simulink model "SIM_EXO_DAL"  (R2021b)
settings: Solver=VariableStepAuto  StartTime=0.0  StopTime=60  FixedStep=0.0001  RelTol=1e-4
undefined symbols (not defined in the file): b, dq, q, X, Y, Z
libraries: sm_lib x47, nesl_utility x7
(part 20 of 25)

== matlab function SIM_EXO_DAL/Energy Analysis/K ==
  data: q input; dq input; K output
function K = K(q,dq)
%#codegen
dq1 = dq(1);
dq2 = dq(2);
dq3 = dq(3);
dq4 = dq(4);
dq5 = dq(5);
dq6 = dq(6);

q1 = q(1);
q2 = q(2);
q3 = q(3);
q4 = q(4);
q5 = q(5);
q6 = q(6);
%    This function was generated by the Symbolic Math Toolbox version 9.0.
%    02-Dec-2021 21:08:55

t2 = cos(q2);
t3 = cos(q4);
t4 = cos(q5);
t5 = cos(q6);
t6 = sin(q2);
t7 = sin(q4);
t8 = sin(q5);
t9 = sin(q6);
t10 = q1+q2;
t11 = q4.*2.0;
t12 = q5.*2.0;
t13 = q6.*2.0;
t30 = 9.007199254740992e+15;
t14 = cos(t12);
t15 = cos(t13);
t16 = t3.^2;
t17 = t4.^2;
t18 = t5.^2;
t19 = sin(t11);
t20 = sin(t12);
t21 = sin(t13);
t22 = cos(t10);
t23 = sin(t10);
t29 = t8.*5.110348748545983e-1;
t31 = t4.*t5.*5.110348748545983e-1;
t32 = t4.*t9.*5.110348748545983e-1;
t33 = t4.*t7.*8.595599785252598e-1;
t34 = t3.*t9.*8.595599785252598e-1;
t35 = t5.*1.33637579258949e-4;
t37 = t3.*t5.*8.595599785252598e-1;
t38 = t9.*7.26350610236655e-5;
t39 = t5.*t7.*t8.*8.595599785252598e-1;
t40 = t7.*t8.*t9.*8.595599785252598e-1;
t41 = t9.*1.744166498897461e-6;
t42 = t5.*1.246862701090643e-6;
t43 = t9.*1.246862701090643e-6;
t44 = t8.*4.20092050615074e-6;
t45 = t5.*3.383302988283333e-6;
t51 = t4.*t9.*3.383302988283333e-6;
t52 = t8.*1.758766830582798e-8;
t53 = t4.*t5.*1.744166498897461e-6;
t54 = t5.*t8.*8.01825475553694e-7;
t55 = t4.*t5.*(-1.246862701090643e-6);
t56 = t4.*t9.*(-1.246862701090643e-6);
t57 = t4.*2.524706033578261e-9;
t58 = t8.*t9.*4.35810366141993e-7;
t59 = t5.*3.146556677756745e-13;
t60 = t8.*3.146556677756745e-13;
t61 = t8.*4.126305279697715e-13;
t62 = t9.*4.126305279697715e-13;
t63 = t4.*t9.*3.146556677756745e-13;
t65 = t4.*t5.*4.126305279697715e-13;
t66 = t5.*t8.*8.4155913e-14;
t67 = t8.*t9.*8.4155913e-14;
t68 = (q3.*t30)./4.503599627370496e+15;
t70 = (q3.*t30)./9.007199254740992e+15;
t78 = t8.*6.829346359246847e-5;
t82 = t3.*5.316841594276996e-5;
t83 = t4.*6.932317328700695e-5;
t84 = t3.*1.166014850920627e-4;
t85 = t3.*t5.*1.148695147579899e-4;
t86 = t8.*3.161026044296245e-5;
t87 = t4.*t9.*6.829346359246847e-5;
t88 = t4.*t7.*1.148695147579899e-4;
t89 = t8.*3.711904932028501e-5;
t90 = t8.*2.146816885134859e-6;
t91 = t8.*3.004073648334264e-7;
t93 = t4.*3.726186752973823e-7;
t94 = t8.*3.726186752973823e-7;
t95 = t4.*t7.*5.316841594276996e-5;
t97 = t4.*3.60334715805357e-7;
t98 = t8.*3.60334715805357e-7;
t99 = t4.*1.153569201933121e-6;
t100 = t7.*t8.*1.166014850920627e-4;
t101 = t3.*2.28624364216682e-6;
t102 = t8.*8.987911871652987e-9;
t103 = t4.*t5.*3.711904932028501e-5;
t104 = t7.*t8.*t9.*1.148695147579899e-4;
t106 = t4.*t7.*6.243419149368285e-5;
t107 = t3.*t9.*6.243419149368285e-5;
t108 = t4.*t5.*8.913299084896471e-7;
t115 = t4.*t9.*1.728985819212562e-6;
t116 = t4.*t5.*6.371903244127231e-7;
t117 = t4.*t9.*6.371903244127231e-7;
t118 = t7.*t8.*1.940301860461398e-6;
t119 = t4.*t7.*3.610943140053254e-6;
t120 = t3.*t5.*2.908151843953269e-6;
t122 = t4.*t7.*5.052847873416058e-7;
t123 = t3.*t5.*1.07175327657342e-6;
t124 = t3.*t9.*1.07175327657342e-6;
t125 = t3.*t9.*1.49921571833678e-6;
t126 = t4.*t7.*6.267441153167058e-7;
t127 = t7.*t8.*6.267441153167058e-7;
t128 = t3.*1.511765579126689e-8;
t129 = t4.*t7.*6.060825118201251e-7;
t131 = t7.*t8.*6.060825118201251e-7;
t134 = t4.*1.290212831914316e-9;
t135 = t8.*1.608000198040319e-13;
t137 = t3.*2.170136264005124e-9;
t140 = t5.*t7.*t8.*6.243419149368285e-5;
t141 = t3.*t4.*t9.*6.892170885479394e-7;
t143 = t7.*t8.*t9.*2.908151843953269e-6;
t144 = t5.*t7.*t8.*1.07175327657342e-6;
t146 = t7.*t8.*t9.*1.07175327657342e-6;
t147 = t5.*t7.*t8.*1.49921571833678e-6;
t149 = t4.*t7.*1.511765579126689e-8;
t150 = t4.*t9.*1.608000198040319e-13;
t153 = t7.*t8.*2.170136264005124e-9;
t154 = t3.*t8.*(-1.511765579126689e-8);
t157 = t3.*t4.*t5.*3.746051489620971e-7;
t158 = t4.*t5.*7.16776774470491e-12;
t159 = t4.*t9.*7.16776774470491e-12;
t160 = t8.*2.10868590222219e-13;
t161 = t3.*t5.*2.7046541903611e-13;
t162 = t4.*t7.*2.7046541903611e-13;
t164 = t3.*t5.*1.205617579517561e-11;
t165 = t3.*t9.*1.205617579517561e-11;
t167 = t4.*t7.*3.546806877605634e-13;
t168 = t3.*t9.*3.546806877605634e-13;
t169 = t4.*t5.*2.10868590222219e-13;
t172 = t7.*t8.*t9.*2.7046541903611e-13;
t173 = t5.*t7.*t8.*1.205617579517561e-11;
t174 = t7.*t8.*t9.*1.205617579517561e-11;
t177 = t5.*t7.*t8.*3.546806877605634e-13;
t180 = t3.*t8.*t9.*(-3.546806877605634e-13);
t192 = t3.*2.625549359694895e-3;
t193 = t4.*1.560969940408669e-3;
t194 = t8.*1.560969940408669e-3;
t195 = t6.*t8.*1.324388487819695e-2;
t196 = t2.*t8.*5.463144604697158e-2;
t202 = t4.*t7.*2.625549359694895e-3;
t204 = t7.*t8.*2.625549359694895e-3;
t207 = t4.*t6.*t7.*2.227619671697157e-2;
t208 = t7.*5.363539617571206e-4;
t209 = t3.*t5.*(-2.625549359694895e-3);
t210 = t4.*t5.*(-1.560969940408669e-3);
t211 = t4.*t9.*(-1.560969940408669e-3);
t217 = t2.*t4.*t7.*9.189001945180305e-2;
t218 = t5.*1.184846851663018e-6;
t223 = t7.*3.050168925520967e-6;
t226 = t7.*6.689201101650821e-6;
t230 = t3.*t4.*5.363539617571206e-4;
t231 = t3.*t8.*5.363539617571206e-4;
t233 = t3.*t9.*6.589841321991422e-6;
t237 = t3.*t4.*3.050168925520967e-6;
t240 = t3.*t8.*6.689201101650821e-6;
t246 = t3.*t8.*1.545129867076994e-8;
t247 = t3.*t4.*t9.*7.044279371874937e-7;
t248 = t9.*6.439911875946239e-7;
t249 = t3.*t5.*3.581728501918121e-6;
t255 = t5.*t7.*t8.*6.589841321991422e-6;
t269 = t3.*t7.*t8.*t9.*4.188040994443703e-7;
t270 = t3.*2.783427048984746e-6;
t271 = t4.*t5.*t7.*t8.*1.408855874374987e-6;
t272 = t3.*t4.*t5.*t9.*1.440030993265091e-6;
t273 = t7.*t8.*t9.*3.581728501918121e-6;
t275 = t3.*t4.*t7.*9.186272837068685e-9;
t280 = t3.*t4.*3.476977846858022e-8;
t281 = t3.*t8.*3.476977846858022e-8;
t282 = t3.*t4.*t5.*3.828725908394669e-7;
t286 = t3.*t5.*t7.*t8.*t9.*8.561427670149984e-7;
t294 = t3.*t5.*t7.*t8.*2.276295446893622e-7;
t302 = t7.*t8.*5.200343311959535e-6;
t303 = t7.*t9.*2.764345231392299e-13;
t306 = t4.*t5.*t7.*t8.*t9.*2.190813206274814e-6;
t308 = t3.*t4.*1.093188572509221e-6;
t311 = t4.*t7.*t8.*t9.*7.657451816789338e-7;
t320 = t3.*t5.*t8.*2.764345231392299e-13;
t328 = t4.*t8.*t9.*3.006136635626675e-13;
t332 = t5.*t7.*3.625084017661248e-13;
t335 = t3.*t7.*t8.*6.499342678834474e-7;
t341 = t3.*t4.*t5.*t7.*1.643488359943407e-13;
t345 = t3.*t8.*t9.*3.625084017661248e-13;
t346 = t4.*t7.*t8.*5.185406908527248e-7;
t348 = t4.*t5.*t8.*3.94216241479634e-13;
t350 = t3.*t4.*t7.*t9.*2.155224072299545e-13;
t360 = t4.*t7.*6.689200410011394e-6;
t379 = t8.*2.086042441322004e-7;
t384 = t8.*1.133811468776912e-7;
t386 = t4.*t9.*2.086042441322004e-7;
t389 = t2.*t4.*t5.*1.769880715106441e-6;
t390 = t4.*t6.*t9.*1.769880715106441e-6;
t391 = t5.*t6.*t8.*1.769880715106441e-6;
t393 = t3.*4.911624408131596e-10;
t394 = t4.*t5.*1.133811468776912e-7;
t396 = t3.*t5.*3.508720606545093e-7;
t399 = t4.*t7.*3.508720606545093e-7;
t400 = t7.*t9.*3.508720606545093e-7;
t401 = t2.*t7.*4.167215943261981e-9;
t402 = t3.*t6.*4.167215943261981e-9;
t403 = t6.*t7.*t9.*2.976937004352228e-6;
t404 = t4.*t5.*1.209061939415321e-5;
t407 = t2.*t4.*t9.*7.30081420113316e-6;
t408 = t2.*t5.*t8.*7.30081420113316e-6;
t409 = t4.*t5.*t6.*7.30081420113316e-6;
t412 = t2.*t3.*t9.*2.976937004352228e-6;
t413 = t3.*t5.*t6.*2.976937004352228e-6;
t416 = t8.*1.646190906295504e-7;
t417 = t2.*t3.*t5.*1.22799597575967e-5;
t418 = t2.*t7.*t9.*1.22799597575967e-5;
t419 = t3.*t6.*t9.*1.22799597575967e-5;
t423 = t3.*t9.*2.033640570959539e-5;
t424 = t4.*t7.*1.907069379620846e-7;
t425 = t3.*t9.*1.907069379620846e-7;
t426 = t5.*t7.*1.907069379620846e-7;
t430 = t6.*t8.*t9.*9.619703863182361e-7;
t431 = t2.*t4.*1.396693317797299e-6;
t432 = t6.*t8.*1.396693317797299e-6;
t433 = t2.*t4.*t5.*3.96815841743287e-6;
t434 = t2.*t8.*t9.*3.96815841743287e-6;
t435 = t4.*t6.*t9.*3.96815841743287e-6;
t436 = t2.*t3.*t5.*1.618032907912407e-6;
t439 = t2.*t3.*1.718989821069714e-8;
t440 = t3.*t6.*t9.*1.618032907912407e-6;
t441 = t5.*t6.*t7.*1.618032907912407e-6;
t442 = t6.*t7.*1.718989821069714e-8;
t443 = t7.*t8.*t9.*(-3.508720606545093e-7);
t445 = t2.*t5.*t7.*t8.*2.976937004352228e-6;
t447 = t4.*t5.*t6.*t7.*2.976937004352228e-6;
t448 = t2.*t4.*t9.*9.619703863182361e-7;
t449 = t4.*t5.*t6.*9.619703863182361e-7;
t451 = t4.*t9.*6.571526380364474e-6;
t453 = t3.*t5.*1.105329861487718e-5;
t455 = t2.*t4.*t5.*t7.*1.22799597575967e-5;
t459 = t5.*t6.*t7.*t8.*1.22799597575967e-5;
t463 = t7.*4.452917654948397e-7;
t464 = t5.*t7.*t8.*2.033640570959539e-5;
t468 = t2.*t8.*5.761404326386517e-6;
t469 = t4.*t6.*5.761404326386517e-6;
t471 = t3.*t5.*t6.*t8.*(-2.976937004352228e-6);
t473 = t2.*t3.*t9.*6.674437170347525e-6;
t474 = t2.*t5.*t7.*6.674437170347525e-6;
t475 = t3.*t5.*t6.*6.674437170347525e-6;
t476 = t4.*9.541257312828922e-6;
t478 = t3.*t8.*2.768890910755245e-7;
t479 = t4.*t7.*2.768890910755245e-7;
t480 = t2.*t3.*3.778031034908185e-6;
t481 = t2.*t7.*t8.*t9.*(-1.22799597575967e-5);
t483 = t6.*t7.*3.778031034908185e-6;
t484 = t2.*t7.*t8.*t9.*1.618032907912407e-6;
t486 = t4.*t6.*t7.*t9.*1.618032907912407e-6;
t490 = t7.*t8.*t9.*1.105329861487718e-5;
t492 = t2.*t7.*t8.*2.349236299369594e-6;
t493 = t3.*t6.*t8.*2.349236299369594e-6;
t494 = t4.*t6.*t7.*2.349236299369594e-6;
t496 = t3.*t6.*t8.*t9.*(-1.618032907912407e-6);
t498 = t5.*t6.*t7.*t8.*(-1.618032907912407e-6);
t499 = t2.*t7.*1.558449809444963e-5;
t500 = t3.*t6.*1.558449809444963e-5;
t502 = t2.*t4.*t7.*t9.*6.674437170347525e-6;
t504 = t6.*t7.*t8.*t9.*6.674437170347525e-6;
t505 = t3.*2.010604972694953e-5;
t513 = t4.*t5.*2.189414175010785e-14;
t514 = t4.*t9.*2.189414175010785e-14;
t515 = t7.*t8.*1.604838208596364e-5;
t516 = t2.*t3.*t8.*9.690674399615435e-6;
t517 = t2.*t4.*t7.*9.690674399615435e-6;
t518 = t6.*t7.*t8.*9.690674399615435e-6;
t519 = t7.*6.664488561844862e-7;
t521 = t3.*t5.*3.682591724861488e-14;
t523 = t3.*t9.*3.682591724861488e-14;
t526 = t5.*t7.*t8.*3.682591724861488e-14;
t527 = t7.*t8.*t9.*3.682591724861488e-14;
t528 = t4.*2.11749498538388e-7;
t536 = t2.*t8.*1.796566294495167e-6;
t537 = t4.*t6.*1.796566294495167e-6;
t541 = t2.*t4.*7.410893064247368e-6;
t542 = t6.*t8.*7.410893064247368e-6;
t544 = t3.*t4.*3.561623743745041e-7;
t545 = t7.*t8.*3.561623743745041e-7;
t546 = t8.*1.227291709418896e-5;
t547 = t2.*t4.*t7.*3.021822113324163e-6;
t548 = t3.*t4.*t6.*3.021822113324163e-6;
t549 = t6.*t7.*t8.*3.021822113324163e-6;
t555 = t4.*t7.*2.06430301981345e-5;
t558 = t2.*t3.*t4.*1.246511225866906e-5;
t559 = t2.*t7.*t8.*1.246511225866906e-5;
t560 = t4.*t6.*t7.*1.246511225866906e-5;
t595 = t2.*1.410504133294943e-4;
t598 = t6.*4.897880306001738e-4;
t24 = t23.*7.742227997977903e+15;
t25 = t22.*4.602992943936994e+15;
t26 = t23.*4.602992943936994e+15;
t27 = t22.*7.742227997977903e+15;
t36 = -t31;
t46 = -t40;
t48 = t4.*t42;
t49 = t4.*t43;
t64 = -t62;
t69 = sin(t68);
t71 = cos(t70);
t72 = sin(t70);
t92 = -t83;
t96 = -t90;
t105 = -t93;
t109 = -t97;
t110 = -t98;
t111 = -t99;
t112 = -t102;
t113 = -t103;
t114 = -t104;
t121 = t29+t33;
t130 = -t116;
t132 = -t117;
t133 = -t119;
t136 = -t123;
t138 = -t125;
t139 = -t128;
t142 = -t129;
t145 = -t134;
t148 = t8.*t128;
t151 = -t143;
t152 = -t147;
t155 = -t149;
t156 = -t150;
t163 = -t157;
t166 = -t161;
t170 = -t165;
t171 = t8.*t161;
t175 = -t169;
t176 = t8.*t168;
t178 = -t173;
t179 = -t174;
t181 = t52+t57;
t182 = t20.*3.726186322907759e-7;
t197 = -t193;
t200 = -t195;
t201 = t5.*t192;
t203 = t9.*t192;
t205 = t5.*t193;
t206 = t9.*t193;
t219 = -t207;
t221 = t5.*t204;
t222 = t9.*t204;
t224 = t18.*4.280713835074992e-7;
t229 = t21.*3.256264776948168e-7;
t251 = t5.*t16.*4.188040994443703e-7;
t253 = t5.*t17.*7.660427522186475e-7;
t257 = t9.*t16.*2.276295446893622e-7;
t258 = t16.*t18.*8.561427670149984e-7;
t260 = t19.*4.420145378913349e-10;
t261 = -t247;
t262 = -t249;
t268 = t5.*t9.*t16.*1.302505910779267e-6;
t276 = t17.*t18.*7.829937223708732e-7;
t277 = t5.*t9.*t17.*1.191219491402018e-6;
t278 = t3.*t4.*t18.*2.190813206274814e-6;
t287 = -t269;
t288 = -t270;
t289 = -t271;
t290 = t9.*t17.*4.163616429052617e-7;
t291 = -t272;
t292 = -t275;
t297 = -t281;
t298 = t3.*t7.*t8.*t18.*1.302505910779267e-6;
t305 = -t286;
t309 = t4.*t7.*t8.*t18.*1.440030993265091e-6;
t315 = -t306;
t316 = -t308;
t321 = -t311;
t322 = t5.*t16.*t17.*(-4.188040994443703e-7);
t324 = t5.*t9.*t16.*t17.*6.512529553896337e-7;
t325 = t16.*1.035461175802946e-6;
t326 = t9.*t16.*t17.*(-2.276295446893622e-7);
t327 = t16.*t17.*t18.*(-4.280713835074992e-7);
t329 = t17.*2.81948171692439e-7;
t331 = -t320;
t338 = t7.*t9.*t17.*5.528690462784599e-13;
t343 = -t335;
t347 = t4.*t8.*t9.*t16.*1.643488359943407e-13;
t349 = t16.*t17.*1.54144203823673e-7;
t351 = -t350;
t352 = t5.*t7.*t17.*7.250168035322496e-13;
t353 = t4.*t5.*t8.*t16.*2.155224072299545e-13;
t355 = t35+t38+4.36041e-5;
t362 = -t360;
t363 = t20.*3.483029800032151e-7;
t364 = t43+t45+8.01825475553694e-7;
t365 = t7.*t17.*1.281152254279884e-6;
t368 = t41+t42+4.35810366141993e-7;
t371 = t4.*t8.*t16.*3.808422322424164e-7;
t387 = t5.*t379;
t395 = t9.*t384;
t397 = -t390;
t398 = -t391;
t406 = -t394;
t411 = -t400;
t414 = -t401;
t415 = -t402;
t420 = t8.*t396;
t421 = t5.*t399;
t422 = t8.*t400;
t428 = -t412;
t429 = -t413;
t437 = -t418;
t438 = -t419;
t444 = -t423;
t446 = t8.*t413;
t450 = t8.*t403;
t452 = -t430;
t454 = t8.*t417;
t456 = -t432;
t457 = -t433;
t458 = t8.*t418;
t460 = -t440;
t461 = -t441;
t462 = -t442;
t465 = t8.*t425;
t466 = t9.*t424;
t467 = t8.*t426;
t470 = -t445;
t472 = -t447;
t482 = -t459;
t485 = t8.*t440;
t487 = t8.*t441;
t488 = -t464;
t491 = -t483;
t495 = -t484;
t497 = -t486;
t501 = t8.*t473;
t503 = t8.*t474;
t507 = -t490;
t508 = -t492;
t509 = -t493;
t510 = -t494;
t511 = -t504;
t520 = -t515;
t522 = -t518;
t524 = -t519;
t525 = -t523;
t533 = -t526;
t534 = -t527;
t535 = -t528;
t543 = -t541;
t550 = -t544;
t556 = -t549;
t562 = -t558;
t714 = t51+t55+t60+t67;
t738 = t53+t56+t61+t66;
t1091 = t44+t54+t58+t63+t65;
t28 = -t26;
t47 = t24+t25;
t73 = t71.^2;
t74 = t3.*t71;
t75 = t7.*t71;
t76 = t71-1.0;
t183 = t71.*2.118754404193375e+31;
t184 = -t182;
t186 = t59+t64;
t189 = t4.*t71.*5.157359871151559e-3;
t232 = -t224;
t234 = -t229;
t267 = -t253;
t295 = -t276;
t296 = -t277;
t307 = -t290;
t312 = t17.*t251;
t317 = t17.*t257;
t318 = t16.*t17.*t224;
t319 = -t309;
t336 = -t324;
t337 = -t325;
t340 = t3.*t30.*t72.*4.602992943936994e+15;
t344 = -t338;
t354 = -t352;
t356 = t34+t36+t39;
t357 = t32+t37+t46;
t361 = t3.*t8.*t30.*t72.*6.661338147750939e-19;
t366 = -t363;
t369 = t71.*7.38843356682345e-1;
t370 = t71.*2.61156643317655e-1;
t372 = t71.*4.392651260556773e-1;
t373 = t71.*4.931128922368695e-2;
t374 = -t371;
t377 = t30.*t72.*8.001214128951626e+33;
t381 = t4.*t30.*t72.*8.368294830410569e+32;
t382 = t7.*t8.*t30.*t72.*4.97520895370488e+32;
t383 = t4.*t71.*1.511765579126689e-8;
t405 = t4.*t16.*t71.*3.023531158253378e-8;
t410 = t16.*t71.*2.909656073620116e-9;
t489 = -t7.*t30.*t72.*(t26-t27);
t512 = t7.*t30.*t72.*(t26-t27);
t529 = t3.*t30.*t72.*5.673626844500105e-17;
t530 = t7.*t30.*t72.*5.673626844500105e-17;
t531 = t4.*t30.*t72.*9.543032792050485e-17;
t532 = t8.*t30.*t72.*9.543032792050485e-17;
t540 = t3.*t30.*t72.*3.404176106700063e-19;
t551 = t5.*t8.*t30.*t72.*5.725819675230291e-19;
t552 = t8.*t9.*t30.*t72.*5.725819675230291e-19;
t553 = t4.*t5.*t7.*t30.*t72.*3.404176106700063e-19;
t554 = t4.*t7.*t9.*t30.*t72.*3.404176106700063e-19;
t563 = t2.*t8.*t71.*2.227619671697157e-2;
t564 = t4.*t71.*5.088811214040866e-2;
t565 = t8.*t71.*5.088811214040866e-2;
t567 = t6.*t8.*t71.*9.189001945180305e-2;
t590 = t2.*t71.*4.472183499114333e-13;
t605 = t6.*t71.*1.844789907123413e-12;
t617 = t71.*1.454432002254732e-9;
t655 = t3.*t30.*t72.*(t26-t27).*(-1.232595164407831e-32);
t668 = t7.*t30.*t72.*9.827649182848514e-18;
K = ft_1({dq1,dq2,dq3,dq4,dq5,dq6,t100,t101,t102,t105,t106,t107,t108,t109,t1091,t110,t111,t112,t113,t114,t115,t118,t119,t120,t121,t122,t124,t126,t127,t130,t131,t132,t133,t135,t136,t137,t138,t139,t14,t140,t141,t142,t144,t145,t146,t15,t150,t151,t152,t153,t154,t155,t156,t158,t159,t16,t160,t161,t162,t163,t164,t166,t167,t168,t169,t17,t170,t171,t172,t175,t177,t178,t179,t18,t180,t181,t183,t184,t186,t189,t19,t192,t194,t196,t197,t2,t20,t200,t202,t203,t204,t208,t209,t21,t210,t211,t217,t218,t219,t22,t221,t222,t223,t226,t23,t230,t231,t232,t233,t234,t237,t240,t246,t247,t248,t251,t253,t255,t257,t258,t26,t260,t261,t262,t267,t268,t27,t271,t272,t273,t276,t277,t278,t28,t280,t282,t287,t288,t289,t290,t291,t292,t294,t295,t296,t297,t298,t3,t30,t302,t303,t305,t306,t307,t308,t309,t311,t315,t316,t319,t320,t321,t322,t326,t327,t328,t329,t331,t332,t336,t337,t338,t340,t341,t343,t344,t345,t346,t347,t348,t349,t35,t351,t352,t353,t354,t355,t356,t357,t361,t362,t364,t365,t366,t368,t369,t370,t372,t373,t374,t377,t379,t38,t381,t382,t383,t384,t386,t387,t389,t391,t393,t395,t396,t397,t398,t399,t4,t403,t404,t405,t406,t407,t408,t409,t41,t410,t411,t414,t415,t416,t417,t42,t420,t421,t424,t425,t426,t428,t429,t43,t430,t431,t432,t434,t435,t436,t437,t438,t439,t443,t444,t448,t449,t45,t450,t451,t452,t453,t454,t455,t456,t457,t460,t461,t462,t463,t465,t466,t467,t468,t469,t47,t470,t471,t472,t473,t474,t475,t476,t478,t479,t480,t481,t482,t488,t491,t495,t496,t497,t498,t499,t5,t500,t501,t502,t503,t505,t507,t508,t509,t510,t511,t512,t513,t514,t516,t517,t52,t520,t521,t522,t523,t524,t525,t526,t529,t530,t531,t532,t533,t534,t535,t536,t537,t540,t541,t542,t543,t545,t546,t547,t548,t550,t551,t552,t553,t554,t555,t556,t559,t560,t562,t563,t564,t565,t567,t59,t590,t595,t598,t6,t605,t61,t617,t62,t655,t668,t69,t7,t71,t714,t72,t73,t738,t74,t75,t76,t78,t8,t82,t84,t85,t86,t87,t88,t89,t9,t90,t91,t92,t94,t95,t96});
end
function K = ft_1(ct)
dq1 = ct{1};
dq2 = ct{2};
dq3 = ct{3};
dq4 = ct{4};
dq5 = ct{5};
dq6 = ct{6};
t100 = ct{7};
t101 = ct{8};
t102 = ct{9};
t105 = ct{10};
t106 = ct{11};
t107 = ct{12};
t108 = ct{13};
t109 = ct{14};
t1091 = ct{15};
t110 = ct{16};
t111 = ct{17};
t112 = ct{18};
t113 = ct{19};
t114 = ct{20};
t115 = ct{21};
t118 = ct{22};
t119 = ct{23};
t120 = ct{24};
t121 = ct{25};
t122 = ct{26};
t124 = ct{27};
t126 = ct{28};
t127 = ct{29};
t130 = ct{30};
t131 = ct{31};
t132 = ct{32};
t133 = ct{33};
t135 = ct{34};
t136 = ct{35};
t137 = ct{36};
t138 = ct{37};
t139 = ct{38};
t14 = ct{39};
t140 = ct{40};
t141 = ct{41};
t142 = ct{42};
t144 = ct{43};
t145 = ct{44};
t146 = ct{45};
t15 = ct{46};
t150 = ct{47};
t151 = ct{48};
t152 = ct{49};
t153 = ct{50};
t154 = ct{51};
t155 = ct{52};
t156 = ct{53};
t158 = ct{54};
t159 = ct{55};
t16 = ct{56};
t160 = ct{57};
t161 = ct{58};
t162 = ct{59};
t163 = ct{60};
t164 = ct{61};
t166 = ct{62};
t167 = ct{63};
t168 = ct{64};
t169 = ct{65};
t17 = ct{66};
t170 = ct{67};
t171 = ct{68};
t172 = ct{69};
t175 = ct{70};
t177 = ct{71};
t178 = ct{72};
t179 = ct{73};
t18 = ct{74};
t180 = ct{75};
t181 = ct{76};
t183 = ct{77};
t184 = ct{78};
t186 = ct{79};
t189 = ct{80};
t19 = ct{81};
t192 = ct{82};
t194 = ct{83};
t196 = ct{84};
t197 = ct{85};
t2 = ct{86};
t20 = ct{87};
t200 = ct{88};
t202 = ct{89};
t203 = ct{90};
t204 = ct{91};
t208 = ct{92};
t209 = ct{93};
t21 = ct{94};
t210 = ct{95};
t211 = ct{96};
t217 = ct{97};
t218 = ct{98};
t219 = ct{99};
t22 = ct{100};
t221 = ct{101};
t222 = ct{102};
t223 = ct{103};
t226 = ct{104};
t23 = ct{105};
t230 = ct{106};
t231 = ct{107};
t232 = ct{108};
t233 = ct{109};
t234 = ct{110};
t237 = ct{111};
t240 = ct{112};
t246 = ct{113};
t247 = ct{114};
t248 = ct{115};
t251 = ct{116};
t253 = ct{117};
t255 = ct{118};
t257 = ct{119};
t258 = ct{120};
t26 = ct{121};
t260 = ct{122};
t261 = ct{123};
t262 = ct{124};
t267 = ct{125};
t268 = ct{126};
t27 = ct{127};
t271 = ct{128};
t272 = ct{129};
t273 = ct{130};
t276 = ct{131};
t277 = ct{132};
t278 = ct{133};
t28 = ct{134};
t280 = ct{135};
t282 = ct{136};
t287 = ct{137};
t288 = ct{138};
t289 = ct{139};
t290 = ct{140};
t291 = ct{141};
t292 = ct{142};
t294 = ct{143};
t295 = ct{144};
t296 = ct{145};
t297 = ct{146};
t298 = ct{147};
t3 = ct{148};
t30 = ct{149};
t302 = ct{150};
t303 = ct{151};
t305 = ct{152};
t306 = ct{153};
t307 = ct{154};
t308 = ct{155};
t309 = ct{156};
t311 = ct{157};
t315 = ct{158};
t316 = ct{159};
t319 = ct{160};
t320 = ct{161};
t321 = ct{162};
t322 = ct{163};
t326 = ct{164};
t327 = ct{165};
t328 = ct{166};
t329 = ct{167};
t331 = ct{168};
t332 = ct{169};
t336 = ct{170};
t337 = ct{171};
t338 = ct{172};
t340 = ct{173};
t341 = ct{174};
t343 = ct{175};
t344 = ct{176};
t345 = ct{177};
t346 = ct{178};
t347 = ct{179};
t348 = ct{180};
t349 = ct{181};
t35 = ct{182};
t351 = ct{183};
t352 = ct{184};
t353 = ct{185};
t354 = ct{186};
t355 = ct{187};
t356 = ct{188};
t357 = ct{189};
t361 = ct{190};
t362 = ct{191};
t364 = ct{192};
t365 = ct{193};
t366 = ct{194};
t368 = ct{195};
t369 = ct{196};
t370 = ct{197};
t372 = ct{198};
t373 = ct{199};
t374 = ct{200};
t377 = ct{201};
t379 = ct{202};
t38 = ct{203};
t381 = ct{204};
t382 = ct{205};
t383 = ct{206};
t384 = ct{207};
t386 = ct{208};
t387 = ct{209};
t389 = ct{210};
t391 = ct{211};
t393 = ct{212};
t395 = ct{213};
t396 = ct{214};
t397 = ct{215};
t398 = ct{216};
t399 = ct{217};
t4 = ct{218};
t403 = ct{219};
t404 = ct{220};
t405 = ct{221};
t406 = ct{222};
t407 = ct{223};
t408 = ct{224};
t409 = ct{225};
t41 = ct{226};
t410 = ct{227};
t411 = ct{228};
t414 = ct{229};
t415 = ct{230};
t416 = ct{231};
t417 = ct{232};
t42 = ct{233};
t420 = ct{234};
t421 = ct{235};
t424 = ct{236};
t425 = ct{237};
t426 = ct{238};
t428 = ct{239};
t429 = ct{240};
t43 = ct{241};
t430 = ct{242};
t431 = ct{243};
t432 = ct{244};
t434 = ct{245};
t435 = ct{246};
t436 = ct{247};
t437 = ct{248};
t438 = ct{249};
t439 = ct{250};
t443 = ct{251};
t444 = ct{252};
t448 = ct{253};
t449 = ct{254};
t45 = ct{255};
t450 = ct{256};
t451 = ct{257};
t452 = ct{258};
t453 = ct{259};
t454 = ct{260};
t455 = ct{261};
t456 = ct{262};
t457 = ct{263};
t460 = ct{264};
t461 = ct{265};
t462 = ct{266};
t463 = ct{267};
t465 = ct{268};
t466 = ct{269};
t467 = ct{270};
t468 = ct{271};
t469 = ct{272};
t47 = ct{273};
t470 = ct{274};
t471 = ct{275};
t472 = ct{276};
t473 = ct{277};
t474 = ct{278};
t475 = ct{279};
t476 = ct{280};
t478 = ct{281};
t479 = ct{282};
t480 = ct{283};
t481 = ct{284};
t482 = ct{285};
t488 = ct{286};
t491 = ct{287};
t495 = ct{288};
t496 = ct{289};
t497 = ct{290};
t498 = ct{291};
t499 = ct{292};
t5 = ct{293};
t500 = ct{294};
t501 = ct{295};
t502 = ct{296};
t503 = ct{297};
t505 = ct{298};
t507 = ct{299};
t508 = ct{300};
t509 = ct{301};
t510 = ct{302};
t511 = ct{303};
t512 = ct{304};
t513 = ct{305};
t514 = ct{306};
t516 = ct{307};
t517 = ct{308};
t52 = ct{309};
t520 = ct{310};
t521 = ct{311};
t522 = ct{312};
t523 = ct{313};
t524 = ct{314};
t525 = ct{315};
t526 = ct{316};
t529 = ct{317};
t530 = ct{318};
t531 = ct{319};
t532 = ct{320};
t533 = ct{321};
t534 = ct{322};
t535 = ct{323};
t536 = ct{324};
t537 = ct{325};
t540 = ct{326};
t541 = ct{327};
t542 = ct{328};
t543 = ct{329};
t545 = ct{330};
t546 = ct{331};
t547 = ct{332};
t548 = ct{333};
t550 = ct{334};
t551 = ct{335};
t552 = ct{336};
t553 = ct{337};
t554 = ct{338};
t555 = ct{339};
t556 = ct{340};
t559 = ct{341};
t560 = ct{342};
t562 = ct{343};
t563 = ct{344};
t564 = ct{345};
t565 = ct{346};
t567 = ct{347};
t59 = ct{348};
t590 = ct{349};
t595 = ct{350};
t598 = ct{351};
t6 = ct{352};
t605 = ct{353};
t61 = ct{354};
t617 = ct{355};
t62 = ct{356};
t655 = ct{357};
t668 = ct{358};
t69 = ct{359};
t7 = ct{360};
t71 = ct{361};
t714 = ct{362};
t72 = ct{363};
t73 = ct{364};
t738 = ct{365};
t74 = ct{366};
t75 = ct{367};
t76 = ct{368};
t78 = ct{369};
t8 = ct{370};
t82 = ct{371};
t84 = ct{372};
t85 = ct{373};
t86 = ct{374};
t87 = ct{375};
t88 = ct{376};
t89 = ct{377};
t9 = ct{378};
t90 = ct{379};
t91 = ct{380};
t92 = ct{381};
t94 = ct{382};
t95 = ct{383};
t96 = ct{384};
t670 = t8.*t30.*t72.*4.008952214699383e-22;
t672 = t2.*t3.*t4.*t30.*t72.*2.877233365226343e-18;
t673 = t3.*t30.*t72.*4.549258542705501e-23;
t674 = t3.*t4.*t6.*t30.*t72.*1.186867907736671e-17;
t676 = t3.*t4.*t30.*t72.*9.827649182848514e-18;
t678 = t3.*t8.*t30.*t72.*9.827649182848514e-18;
t681 = t5.*t30.*t72.*1.530369361342075e-22;
t683 = t7.*t9.*t30.*t72.*(-9.827649182848514e-18);
t684 = t3.*t5.*t30.*t72.*9.098517085411002e-23;
t687 = t3.*t30.*t72.*2.472625392454631e-23;
t688 = t3.*t5.*t9.*t30.*t72.*1.414846738462756e-22;
t689 = t8.*t30.*t72.*1.678396953782234e-24;
t690 = t3.*t9.*t30.*t72.*4.945250784909262e-23;
t691 = t9.*t30.*t72.*8.317905230417136e-23;
t693 = t4.*t5.*t7.*t30.*t72.*4.549258542705501e-23;
t694 = t7.*t8.*t9.*t30.*t72.*4.549258542705501e-23;
t695 = t3.*t18.*t30.*t72.*9.299848787979342e-23;
t696 = t4.*t9.*t30.*t72.*7.651846806710377e-23;
t697 = t5.*t8.*t30.*t72.*7.651846806710377e-23;
t698 = t3.*t8.*t30.*t72.*9.978586703210931e-25;
t699 = t4.*t7.*t30.*t72.*9.978586703210931e-25;
t702 = t4.*t18.*t30.*t72.*2.379770328738529e-22;
t703 = t3.*t4.*t9.*t30.*t72.*(-4.549258542705501e-23);
t707 = t4.*t5.*t9.*t30.*t72.*1.564233326885588e-22;
t709 = t5.*t17.*t30.*t72.*(-1.530369361342075e-22);
t710 = t3.*t4.*t5.*t9.*t30.*t72.*9.299848787979342e-23;
t711 = t5.*t7.*t8.*t9.*t30.*t72.*9.299848787979342e-23;
t712 = t4.*t5.*t30.*t72.*4.158952615208568e-23;
t713 = t8.*t9.*t30.*t72.*4.158952615208568e-23;
t715 = t4.*t5.*t7.*t8.*t30.*t72.*9.098517085411002e-23;
t716 = t3.*t4.*t18.*t30.*t72.*1.414846738462756e-22;
t717 = t7.*t8.*t18.*t30.*t72.*1.414846738462756e-22;
t719 = t7.*t9.*t30.*t72.*1.785238843466173e-29;
t722 = t8.*t30.*t72.*3.002769355787804e-29;
t724 = t4.*t7.*t9.*t30.*t72.*2.472625392454631e-23;
t725 = t5.*t7.*t8.*t30.*t72.*2.472625392454631e-23;
t726 = t5.*t9.*t17.*t30.*t72.*2.379770328738529e-22;
t728 = t17.*t18.*t30.*t72.*1.564233326885588e-22;
t729 = t4.*t5.*t7.*t8.*t9.*t30.*t72.*1.414846738462756e-22;
t731 = t4.*t7.*t8.*t9.*t30.*t72.*4.945250784909262e-23;
t734 = t4.*t7.*t8.*t18.*t30.*t72.*9.299848787979342e-23;
t735 = t4.*t30.*t72.*1.187475829122392e-22;
t737 = t3.*t4.*t30.*t72.*7.059909452387201e-23;
t740 = t7.*t8.*t30.*t72.*7.059909452387201e-23;
t746 = t30.*t72.*8.730562784510963e-22;
t750 = t9.*t17.*t30.*t72.*(-8.317905230417136e-23);
t751 = t3.*t5.*t8.*t30.*t72.*1.785238843466173e-29;
t752 = t4.*t5.*t7.*t30.*t72.*1.785238843466173e-29;
t754 = t8.*t30.*t72.*3.937746659416635e-29;
t755 = t4.*t8.*t9.*t30.*t72.*6.005538711575609e-29;
t756 = t5.*t8.*t30.*t72.*(-3.002769355787804e-29);
t757 = t30.*t69.*9.59842590807046e-26;
t760 = t17.*t30.*t72.*5.632647031707275e-23;
t762 = t3.*t30.*t72.*2.647073057000717e-22;
t763 = t4.*t5.*t71.*7.017441213090186e-7;
t766 = t7.*t9.*t17.*t30.*t72.*3.570477686932346e-29;
t768 = t5.*t7.*t30.*t72.*2.341111640349547e-29;
t774 = t4.*t7.*t8.*t30.*t72.*3.34878210114812e-23;
t775 = t8.*t71.*6.800564119502148e-6;
t782 = t4.*t9.*t71.*3.814138759241691e-7;
t784 = t2.*t4.*t9.*t71.*2.976937004352228e-6;
t785 = t2.*t5.*t8.*t71.*2.976937004352228e-6;
t786 = t4.*t5.*t6.*t71.*2.976937004352228e-6;
t787 = t5.*t8.*t30.*t72.*8.031026374039477e-30;
t788 = t8.*t9.*t30.*t72.*8.031026374039477e-30;
t791 = t4.*t5.*t8.*t30.*t72.*7.875493318833269e-29;
t793 = t3.*t8.*t9.*t30.*t72.*2.341111640349547e-29;
t794 = t4.*t7.*t9.*t30.*t72.*2.341111640349547e-29;
t800 = t8.*t71.*3.696261130697717e-6;
t801 = t5.*t7.*t17.*t30.*t72.*4.682223280699094e-29;
t806 = t4.*t9.*t71.*6.800564119502148e-6;
t819 = t2.*t4.*t5.*t71.*1.22799597575967e-5;
t820 = t4.*t5.*t7.*t30.*t72.*4.774692471202153e-30;
t823 = t4.*t7.*t9.*t30.*t72.*4.774692471202153e-30;
t826 = t4.*t6.*t9.*t71.*1.22799597575967e-5;
t827 = t5.*t6.*t8.*t71.*1.22799597575967e-5;
t836 = t5.*t8.*t71.*(-6.800564119502148e-6);
t839 = t4.*t71.*5.537781821510491e-7;
t845 = t2.*t4.*t5.*t71.*1.618032907912407e-6;
t849 = t2.*t8.*t9.*t71.*1.618032907912407e-6;
t850 = t4.*t6.*t9.*t71.*1.618032907912407e-6;
t855 = t2.*t4.*t9.*t71.*6.674437170347525e-6;
t856 = t4.*t5.*t6.*t71.*6.674437170347525e-6;
t857 = t6.*t8.*t9.*t71.*6.674437170347525e-6;
t869 = t4.*t5.*t71.*3.696261130697717e-6;
t872 = t2.*t8.*t71.*2.349236299369594e-6;
t873 = t4.*t6.*t71.*2.349236299369594e-6;
t896 = t8.*t9.*t71.*(-3.696261130697717e-6);
t901 = t2.*t4.*t71.*9.690674399615435e-6;
t904 = t6.*t8.*t71.*9.690674399615435e-6;
t912 = t8.*t71.*5.366634249353632e-6;
t917 = t7.*t17.*t30.*t72.*8.273795699471084e-23;
t919 = t4.*t8.*t30.*t72.*1.391651334125335e-22;
t925 = t4.*t5.*t71.*7.137559230037459e-13;
t926 = t4.*t9.*t71.*7.137559230037459e-13;
t932 = t8.*t71.*7.123247487490083e-7;
t943 = t2.*t4.*t71.*3.021822113324163e-6;
t944 = t6.*t8.*t71.*3.021822113324163e-6;
t945 = t2.*t8.*t71.*1.246511225866906e-5;
t946 = t4.*t6.*t71.*1.246511225866906e-5;
t950 = t4.*t71.*6.903100404659751e-6;
t967 = t7.*t9.*t30.*t72.*9.063852440050829e-23;
t972 = t3.*t30.*t72.*1.268788366711598e-25;
t973 = t16.*t30.*t72.*1.458099973297124e-22;
t974 = t2.*t3.*t9.*t30.*t72.*3.84506501891928e-22;
t975 = t2.*t5.*t7.*t30.*t72.*3.84506501891928e-22;
t976 = t5.*t7.*t30.*t72.*4.926409762458377e-23;
t977 = t6.*t7.*t9.*t30.*t72.*3.84506501891928e-22;
t978 = t2.*t7.*t30.*t72.*5.382450561195517e-25;
t979 = t3.*t6.*t30.*t72.*5.382450561195517e-25;
t980 = t3.*t5.*t8.*t30.*t72.*9.063852440050829e-23;
t981 = t2.*t7.*t9.*t30.*t72.*1.586101540900623e-21;
t982 = t3.*t6.*t9.*t30.*t72.*1.586101540900623e-21;
t983 = t5.*t6.*t7.*t30.*t72.*1.586101540900623e-21;
t986 = t3.*t4.*t30.*t72.*1.313343246602064e-21;
t987 = t3.*t9.*t30.*t72.*1.313343246602064e-21;
t988 = t5.*t7.*t30.*t72.*1.313343246602064e-21;
t991 = t2.*t3.*t4.*t5.*t30.*t72.*3.84506501891928e-22;
t992 = t2.*t3.*t5.*t30.*t72.*2.089880210625419e-22;
t998 = t3.*t5.*t6.*t8.*t30.*t72.*3.84506501891928e-22;
t999 = t2.*t7.*t9.*t30.*t72.*2.089880210625419e-22;
t1000 = t5.*t6.*t7.*t30.*t72.*2.089880210625419e-22;
t1001 = t3.*t8.*t9.*t30.*t72.*4.926409762458377e-23;
t1004 = t2.*t3.*t30.*t72.*2.220277963292577e-24;
t1005 = t6.*t7.*t30.*t72.*2.220277963292577e-24;
t1006 = t7.*t9.*t30.*t72.*7.138318981153782e-22;
t1009 = t2.*t3.*t8.*t9.*t30.*t72.*(-3.84506501891928e-22);
t1010 = t2.*t5.*t7.*t8.*t30.*t72.*(-3.84506501891928e-22);
t1014 = t2.*t5.*t7.*t30.*t72.*8.620822290548326e-22;
t1015 = t3.*t5.*t6.*t30.*t72.*8.620822290548326e-22;
t1016 = t6.*t7.*t9.*t30.*t72.*8.620822290548326e-22;
t1018 = t3.*t8.*t30.*t72.*9.32742268839803e-25;
t1021 = t30.*t72.*1.170412585872218e-29;
t1022 = t3.*t7.*t30.*t72.*1.650830280755386e-25;
t1023 = t3.*t4.*t30.*t72.*7.138318981153782e-22;
t1024 = t3.*t5.*t30.*t72.*7.138318981153782e-22;
t1025 = t2.*t3.*t5.*t8.*t30.*t72.*1.586101540900623e-21;
t1026 = t3.*t4.*t5.*t6.*t30.*t72.*1.586101540900623e-21;
t1028 = t6.*t30.*t72.*4.965121091065431e-29;
t1029 = t2.*t3.*t4.*t9.*t30.*t72.*2.089880210625419e-22;
t1032 = t3.*t6.*t8.*t9.*t30.*t72.*(-1.586101540900623e-21);
t1033 = t5.*t6.*t7.*t8.*t30.*t72.*(-1.586101540900623e-21);
t1034 = t3.*t8.*t30.*t72.*7.152697935215594e-23;
t1036 = t3.*t6.*t8.*t9.*t30.*t72.*2.089880210625419e-22;
t1037 = t3.*t4.*t7.*t30.*t72.*1.715438754464886e-24;
t1039 = t3.*t8.*t9.*t30.*t72.*(-1.313343246602064e-21);
t1040 = t5.*t7.*t8.*t30.*t72.*(-1.313343246602064e-21);
t1041 = t7.*t30.*t72.*1.150293599235621e-22;
t1043 = t3.*t30.*t72.*1.298466651472986e-21;
t1044 = t2.*t7.*t30.*t72.*2.01292161617043e-21;
t1045 = t3.*t6.*t30.*t72.*2.01292161617043e-21;
t1046 = t2.*t7.*t8.*t9.*t30.*t72.*(-2.089880210625419e-22);
t1048 = t2.*t3.*t8.*t9.*t30.*t72.*8.620822290548326e-22;
t1049 = t3.*t4.*t6.*t9.*t30.*t72.*8.620822290548326e-22;
t1051 = t2.*t3.*t4.*t30.*t72.*3.034315574254804e-22;
t1053 = t2.*t3.*t30.*t72.*4.879772380631159e-22;
t1055 = t2.*t7.*t8.*t30.*t72.*3.034315574254804e-22;
t1056 = t3.*t6.*t8.*t30.*t72.*3.034315574254804e-22;
t1057 = t6.*t7.*t30.*t72.*4.879772380631159e-22;
t1060 = t2.*t30.*t72.*2.048128230484517e-28;
t1062 = t6.*t7.*t8.*t9.*t30.*t72.*(-8.620822290548326e-22);
t1066 = t7.*t8.*t9.*t30.*t72.*(-7.138318981153782e-22);
t1067 = t2.*t3.*t8.*t30.*t72.*1.251664818208198e-21;
t1068 = t3.*t4.*t6.*t30.*t72.*1.251664818208198e-21;
t1069 = t6.*t7.*t8.*t30.*t72.*1.251664818208198e-21;
t1070 = t3.*t4.*t30.*t72.*1.036418850630278e-21;
t1071 = t7.*t8.*t30.*t72.*1.036418850630278e-21;
t1072 = t71.*1.130782628318448e-5;
t1075 = t7.*t30.*t72.*4.303986245035329e-23;
t1076 = t6.*t71.*4.797002992829487e-5;
t1077 = t5.*t7.*t30.*t72.*1.378424649377201e-28;
t1078 = t7.*t9.*t30.*t72.*1.378424649377201e-28;
t1081 = t2.*t71.*1.978778980640035e-4;
t1083 = t3.*t5.*t8.*t30.*t72.*1.378424649377201e-28;
t1084 = t3.*t8.*t9.*t30.*t72.*1.378424649377201e-28;
t1089 = t3.*t4.*t30.*t72.*9.200513714334576e-23;
t1093 = t2.*t3.*t8.*t30.*t72.*3.903039427556764e-22;
t1094 = t2.*t4.*t7.*t30.*t72.*3.903039427556764e-22;
t1095 = t3.*t4.*t6.*t30.*t72.*3.903039427556764e-22;
t1096 = t2.*t3.*t4.*t30.*t72.*1.610016168721029e-21;
t1097 = t3.*t6.*t8.*t30.*t72.*1.610016168721029e-21;
t1098 = t4.*t6.*t7.*t30.*t72.*1.610016168721029e-21;
t1100 = t3.*t8.*t30.*t72.*1.333145329970004e-21;
t1101 = t4.*t7.*t30.*t72.*1.333145329970004e-21;
t1104 = t8.*t9.*t30.*t71.*t72.*9.098517085411002e-23;
t1105 = t4.*t30.*t71.*t72.*1.995717340642186e-24;
t1109 = t8.*t18.*t30.*t71.*t72.*2.829693476925513e-22;
t1110 = t5.*t8.*t9.*t30.*t71.*t72.*1.859969757595868e-22;
t1111 = t5.*t8.*t30.*t71.*t72.*4.945250784909262e-23;
t1118 = t8.*t30.*t71.*t72.*1.41198189047744e-22;
t1119 = t8.*t9.*t16.*t30.*t71.*t72.*1.8197034170822e-22;
t1120 = t16.*t30.*t71.*t72.*3.841105500485731e-25;
t1121 = t4.*t16.*t30.*t71.*t72.*3.991434681284372e-24;
t1124 = t4.*t5.*t30.*t71.*t72.*3.570477686932346e-29;
t1126 = t8.*t16.*t18.*t30.*t71.*t72.*5.659386953851025e-22;
t1128 = t2.*t7.*t30.*t72.*2.750619948951613e-25;
t1131 = t3.*t30.*t72.*3.977152348965926e-22;
t1133 = t5.*t8.*t16.*t30.*t71.*t72.*9.890501569818525e-23;
t1138 = t6.*t7.*t30.*t72.*1.134639471113644e-24;
t1139 = t5.*t8.*t9.*t16.*t30.*t71.*t72.*3.719939515191737e-22;
t1146 = t7.*t30.*t72.*2.158461812807145e-25;
t1148 = t4.*t9.*t30.*t71.*t72.*4.682223280699094e-29;
t1151 = t8.*t16.*t30.*t71.*t72.*2.82396378095488e-22;
t1160 = t4.*t5.*t16.*t30.*t71.*t72.*7.140955373864693e-29;
t1166 = t3.*t30.*t72.*3.979383867109492e-22;
t1179 = t4.*t9.*t16.*t30.*t71.*t72.*9.364446561398189e-29;
t1195 = t30.*t72.*8.661231089831981e-21;
t1204 = t82+t109+t131+t230;
t1205 = t84+t110+t142+t231;
t1217 = t86+t92+t95+t100+t208;
t1268 = t94+t111+t118+t126+t137+t226+t280;
t1269 = t91+t105+t122+t127+t139+t223+t297;
t1270 = t101+t112+t145+t153+t155+t237+t240;
t50 = t27+t28;
t77 = t75.*(3.0./5.0e+2);
t79 = t4.*t5.*t74.*(3.0./5.0e+2);
t80 = t4.*t9.*t74.*(3.0./5.0e+2);
t185 = t75.*8.112963841460668e+31;
t187 = t22.*t76.*3.563742084504373e+31;
t188 = t23.*t76.*3.563742084504373e+31;
t190 = t8.*t75.*3.06620924912759e-3;
t191 = t75.*8.01825475553694e-7;
t198 = t75.*4.35810366141993e-7;
t199 = t5.*t75.*1.603650951107388e-6;
t212 = t18.*t75.*1.639136489385872e-6;
t213 = t52.*t75;
t214 = t9.*t75.*8.71620732283986e-7;
t215 = t8.*t9.*t74.*8.01825475553694e-7;
t220 = t5.*t9.*t75.*2.493725402181286e-6;
t225 = t4.*t74.*1.758766830582798e-8;
t227 = t4.*t5.*t74.*8.01825475553694e-7;
t228 = t4.*t9.*t75.*(-8.01825475553694e-7);
t235 = t5.*t8.*t9.*t74.*1.639136489385872e-6;
t236 = t4.*t5.*t9.*t75.*1.639136489385872e-6;
t238 = t8.*t18.*t74.*2.493725402181286e-6;
t239 = t4.*t18.*t75.*2.493725402181286e-6;
t241 = t4.*t9.*t74.*4.35810366141993e-7;
t242 = t5.*t8.*t74.*4.35810366141993e-7;
t244 = t4.*t5.*t8.*t74.*1.603650951107388e-6;
t245 = t9.*t74.*3.146556677756745e-13;
t256 = t4.*t5.*t8.*t9.*t74.*2.493725402181286e-6;
t263 = t8.*t74.*1.244337995057065e-6;
t264 = t4.*t75.*1.244337995057065e-6;
t265 = t4.*t8.*t18.*t74.*1.639136489385872e-6;
t266 = t4.*t8.*t9.*t74.*8.71620732283986e-7;
t274 = t75.*4.665574824623396e-6;
t283 = t5.*t74.*4.126305279697715e-13;
t284 = t4.*t59.*t74;
t285 = t8.*t59.*t75;
t293 = t9.*t17.*t74.*6.293113355513489e-13;
t300 = t4.*t8.*t74.*5.902365793397849e-7;
t301 = t4.*t5.*t74.*(-3.146556677756745e-13);
t304 = t5.*t8.*t75.*(-3.146556677756745e-13);
t310 = t4.*t62.*t74;
t313 = t9.*t61.*t75;
t323 = t5.*t17.*t74.*8.252610559395431e-13;
t330 = t8.*t74.*8.769009823985418e+48;
t333 = t4.*t5.*t74.*8.4155913e-14;
t334 = t4.*t9.*t74.*8.4155913e-14;
t358 = t17.*t74.*1.458290424491263e-6;
t367 = t183+5.994209437267293e+31;
t380 = t7.*t74.*2.569961002476882e-6;
t385 = t75.*t102;
t388 = -t383;
t392 = t8.*t75.*(-8.987911871652987e-9);
t427 = -t410;
t477 = t7.*t30.*t47.*t72;
t538 = -t530;
t539 = -t531;
t557 = -t551;
t561 = -t554;
t566 = t74.*8.76226105503051e-2;
t568 = -t563;
t569 = -t565;
t570 = t2.*t4.*t75.*1.324388487819695e-2;
t571 = -t567;
t572 = t4.*t6.*t75.*5.463144604697158e-2;
t574 = t4.*t75.*8.76226105503051e-2;
t576 = t8.*t75.*8.76226105503051e-2;
t577 = t5.*t564;
t578 = t9.*t564;
t579 = t5.*t73.*4.188040994443703e-7;
t580 = t5.*t74.*(-8.76226105503051e-2);
t581 = t75.*1.16331319921549e-5;
t584 = t9.*t73.*2.276295446893622e-7;
t585 = t2.*t74.*4.848080468348049e-9;
t586 = t18.*t73.*2.067207872893371e-6;
t587 = t5.*t9.*t73.*3.144978357570919e-6;
t588 = t74.*1.504998469620115e-8;
t589 = t73.*t253;
t591 = t73.*t246;
t592 = t73.*t247;
t593 = t6.*t74.*1.999848601628674e-8;
t594 = t5.*t16.*t73.*2.022455050551758e-6;
t596 = t3.*t8.*t73.*(-1.545129867076994e-8);
t597 = t75.*1.169554785545351e-5;
t599 = t73.*t276;
t600 = t73.*t277;
t601 = t73.*t278;
t603 = t73.*t282;
t604 = t73.*t271;
t607 = t73.*t272;
t608 = t3.*t4.*t7.*t73.*4.436160944872465e-8;
t609 = t3.*t4.*t18.*t73.*(-2.190813206274814e-6);
t610 = t3.*t4.*t5.*t73.*(-3.828725908394669e-7);
t611 = t16.*t18.*t73.*4.134415745786742e-6;
t612 = t73.*t303;
t613 = t5.*t9.*t16.*t73.*6.289956715141839e-6;
t614 = t3.*t7.*t8.*t9.*t73.*2.022455050551758e-6;
t615 = t73.*t290;
t616 = t3.*t7.*t73.*4.269082063722138e-9;
t618 = t73.*t309;
t619 = t73.*t311;
t621 = t9.*t16.*t73.*1.099250276973348e-6;
t622 = t7.*t9.*t73.*(-2.764345231392299e-13);
t624 = t73.*t306;
t626 = t73.*t308;
t627 = t73.*t320;
t629 = t3.*t5.*t7.*t8.*t9.*t73.*4.134415745786742e-6;
t630 = t3.*t7.*t8.*t18.*t73.*6.289956715141839e-6;
t632 = t73.*t328;
t633 = t73.*t329;
t634 = t73.*t332;
t636 = t3.*t5.*t7.*t8.*t73.*1.099250276973348e-6;
t637 = t4.*t8.*t9.*t73.*(-3.006136635626675e-13);
t638 = t17.*t73.*(-2.81948171692439e-7);
t639 = t5.*t7.*t73.*(-3.625084017661248e-13);
t640 = t3.*t7.*t8.*t73.*3.138610257997577e-6;
t642 = t73.*t338;
t645 = t3.*t4.*t5.*t7.*t73.*7.936601715456896e-13;
t646 = t73.*t345;
t647 = t73.*t346;
t648 = (t3.*t30.*t47.*t72)./8.112963841460668e+31;
t651 = t73.*t348;
t653 = t3.*t8.*t9.*t73.*(-3.625084017661248e-13);
t654 = t4.*t7.*t8.*t73.*(-5.185406908527248e-7);
t656 = t16.*t73.*5.00036577347567e-6;
t658 = t512.*(-1.232595164407831e-32);
t659 = t4.*t5.*t8.*t73.*(-3.94216241479634e-13);
t660 = t73.*t352;
t661 = t4.*t8.*t9.*t16.*t73.*7.936601715456896e-13;
t662 = t512./8.112963841460668e+31;
t663 = t16.*t17.*t73.*7.443807831634578e-7;
t666 = t3.*t4.*t7.*t9.*t73.*1.040783463169498e-12;
t667 = t4.*t5.*t8.*t16.*t73.*1.040783463169498e-12;
t671 = -t668;
t675 = t4.*t8.*t73.*6.966059600064303e-7;
t677 = t73.*t365;
t679 = t5.*t668;
t680 = t9.*t668;
t682 = t7.*t17.*t73.*(-1.281152254279884e-6);
t685 = t5.*t678;
t686 = t9.*t678;
t692 = t4.*t9.*t673;
t700 = t17.*t681;
t701 = t4.*t8.*t16.*t73.*1.83913265673368e-6;
t704 = -t693;
t705 = -t694;
t706 = -t696;
t708 = -t699;
t718 = -t707;
t720 = -t710;
t721 = -t711;
t723 = t4.*t5.*t687;
t727 = -t715;
t730 = -t722;
t732 = -t724;
t733 = -t726;
t736 = -t728;
t739 = t17.*t691;
t741 = -t729;
t742 = t5.*t722;
t743 = -t731;
t744 = t369+2.61156643317655e-1;
t745 = t370+7.38843356682345e-1;
t747 = -t734;
t748 = -t735;
t749 = -t737;
t753 = -t740;
t758 = t9.*t74.*4.172084882644007e-7;
t759 = t372-4.392651260556773e-1;
t761 = -t751;
t764 = t2.*t9.*t75.*1.769880715106441e-6;
t765 = t6.*t9.*t74.*1.769880715106441e-6;
t767 = t9.*t754;
t769 = t2.*t5.*t74.*1.769880715106441e-6;
t772 = t5.*t8.*t75.*4.172084882644007e-7;
t773 = -t766;
t776 = t5.*t74.*2.267622937553823e-7;
t777 = t75.*5.84022389932283e-10;
t779 = t75.*t391;
t780 = t2.*t9.*t74.*7.30081420113316e-6;
t781 = t5.*t6.*t74.*7.30081420113316e-6;
t783 = t6.*t9.*t75.*7.30081420113316e-6;
t789 = -t775;
t790 = t2.*t74.*2.477538195427268e-9;
t792 = t6.*t75.*2.477538195427268e-9;
t797 = t75.*t389;
t798 = t2.*t8.*t9.*t75.*(-1.769880715106441e-6);
t799 = t5.*t6.*t8.*t75.*(-1.769880715106441e-6);
t803 = -t784;
t804 = -t785;
t805 = -t786;
t807 = t5.*t775;
t812 = -t788;
t813 = t3.*t9.*t73.*6.735277470591094e-6;
t814 = t2.*t75.*1.021992379861453e-8;
t815 = t6.*t74.*1.021992379861453e-8;
t816 = t5.*t74.*1.170967356229242e-5;
t818 = t4.*t75.*1.170967356229242e-5;
t821 = t9.*t75.*1.170967356229242e-5;
t822 = t4.*t5.*t73.*1.132872773043163e-5;
t824 = -t794;
t825 = t8.*t9.*t75.*2.267622937553823e-7;
t828 = -t800;
t830 = -t801;
t831 = t2.*t9.*t74.*9.619703863182361e-7;
t832 = t2.*t5.*t75.*9.619703863182361e-7;
t833 = t5.*t6.*t74.*9.619703863182361e-7;
t835 = -t806;
t838 = t74.*5.29479332073745e-7;
t840 = t2.*t5.*t74.*3.96815841743287e-6;
t841 = -t820;
t843 = t6.*t9.*t74.*3.96815841743287e-6;
t844 = t5.*t6.*t75.*3.96815841743287e-6;
t846 = t3.*t5.*t73.*3.660776353481749e-6;
t847 = -t826;
t848 = -t827;
t851 = t75.*t408;
t853 = t75.*t409;
t854 = t6.*t8.*t9.*t75.*(-7.30081420113316e-6);
t858 = t5.*t7.*t8.*t73.*6.735277470591094e-6;
t861 = t4.*t75.*6.364473664374288e-6;
t862 = t9.*t74.*6.364473664374288e-6;
t863 = t5.*t75.*6.364473664374288e-6;
t864 = t8.*t75.*3.292381812591008e-7;
t871 = t4.*t9.*t73.*6.157420948384101e-6;
t874 = t9.*t800;
t875 = -t849;
t876 = -t850;
t878 = t75.*t448;
t880 = t75.*t430;
t881 = -t857;
t882 = t2.*t8.*t74.*1.396693317797299e-6;
t883 = t75.*t431;
t885 = t75.*t432;
t886 = t2.*t75.*2.246155783606385e-6;
t887 = t6.*t74.*2.246155783606385e-6;
t888 = t8.*t9.*t75.*(-1.170967356229242e-5);
t889 = t75.*t434;
t891 = t75.*t435;
t893 = t7.*t8.*t9.*t73.*3.660776353481749e-6;
t894 = -t872;
t895 = -t873;
t897 = t75.*t468;
t898 = t6.*t8.*t74.*5.761404326386517e-6;
t899 = t75.*t469;
t900 = t3.*t73.*2.844856587289647e-6;
t902 = t6.*t8.*t9.*t75.*(-9.619703863182361e-7);
t903 = t4.*t73.*8.940013971103833e-6;
t908 = t75.*8.369355329119605e-6;
t909 = t6.*t8.*t75.*(-1.396693317797299e-6);
t910 = t2.*t74.*9.26546399593074e-6;
t911 = t6.*t75.*9.26546399593074e-6;
t914 = -t904;
t916 = -t912;
t918 = t7.*t8.*t73.*5.315113587256377e-6;
t920 = t8.*t74.*9.240635641966378e-6;
t921 = t4.*t75.*9.240635641966378e-6;
t922 = t74.*7.425831767740348e-7;
t923 = t7.*t73.*6.474095421643823e-7;
t924 = -t919;
t927 = t5.*t74.*1.228993465050726e-12;
t928 = t9.*t74.*1.228993465050726e-12;
t929 = -t925;
t930 = -t926;
t933 = t5.*t8.*t75.*1.228993465050726e-12;
t934 = t8.*t9.*t75.*1.228993465050726e-12;
t935 = t4.*t75.*4.23498997076776e-7;
t940 = t2.*t4.*t74.*1.796566294495167e-6;
t941 = t75.*t536;
t942 = t75.*t537;
t947 = t8.*t73.*1.14995379215611e-5;
t948 = t75+t529;
t951 = -t944;
t953 = t75.*t541;
t954 = t4.*t6.*t74.*7.410893064247368e-6;
t956 = t75.*t542;
t957 = t4.*t74.*1.188622750787503e-5;
t958 = t8.*t75.*1.188622750787503e-5;
t959 = t2.*t4.*t75.*(-7.410893064247368e-6);
t962 = t4.*t7.*t73.*6.836829388815e-6;
t970 = -t967;
t984 = -t974;
t985 = -t975;
t989 = -t978;
t990 = -t979;
t993 = -t981;
t994 = -t982;
t995 = -t983;
K = ft_2({dq1,dq2,dq3,dq4,dq5,dq6,t1000,t1001,t1004,t1005,t1006,t1009,t1010,t1014,t1015,t1016,t1018,t1021,t1022,t1023,t1024,t1025,t1026,t1028,t1029,t1032,t1033,t1034,t1036,t1037,t1039,t1040,t1041,t1043,t1044,t1045,t1046,t1048,t1049,t1051,t1053,t1055,t1056,t1057,t106,t1060,t1062,t1066,t1067,t1068,t1069,t107,t1070,t1071,t1072,t1075,t1076,t1077,t1078,t108,t1081,t1083,t1084,t1089,t1091,t1093,t1094,t1095,t1096,t1097,t1098,t1100,t1101,t1104,t1105,t1109,t1110,t1111,t1118,t1119,t1120,t1121,t1124,t1126,t1128,t113,t1131,t1133,t1138,t1139,t114,t1146,t1148,t115,t1151,t1160,t1166,t1179,t119,t1195,t120,t1204,t1205,t121,t1217,t124,t1268,t1269,t1270,t130,t132,t133,t135,t136,t138,t14,t140,t141,t144,t146,t15,t150,t151,t152,t154,t156,t158,t159,t16,t160,t161,t162,t163,t164,t166,t167,t168,t169,t17,t170,t171,t172,t175,t177,t178,t179,t18,t180,t181,t184,t185,t186,t187,t188,t189,t19,t190,t191,t192,t194,t196,t197,t198,t199,t2,t20,t200,t202,t203,t204,t209,t21,t210,t211,t212,t213,t214,t215,t217,t218,t219,t22,t220,t221,t222,t225,t227,t228,t23,t232,t233,t234,t235,t236,t238,t239,t241,t242,t244,t245,t246,t248,t251,t255,t256,t257,t258,t26,t260,t261,t262,t263,t264,t265,t266,t267,t268,t27,t273,t274,t278,t282,t283,t287,t288,t289,t291,t292,t293,t294,t295,t296,t298,t3,t30,t300,t301,t302,t303,t304,t305,t307,t310,t313,t315,t316,t319,t321,t322,t323,t326,t327,t328,t329,t330,t331,t332,t333,t334,t336,t337,t340,t341,t343,t344,t345,t346,t347,t348,t349,t35,t351,t353,t354,t355,t356,t357,t358,t361,t362,t364,t365,t366,t367,t368,t373,t374,t377,t379,t38,t380,t381,t382,t384,t386,t387,t388,t389,t392,t393,t395,t396,t397,t398,t399,t4,t403,t404,t405,t406,t407,t408,t409,t41,t410,t411,t414,t415,t416,t417,t42,t420,t421,t424,t425,t426,t427,t428,t429,t43,t431,t434,t435,t436,t437,t438,t439,t443,t444,t448,t449,t45,t450,t451,t452,t453,t454,t455,t456,t457,t460,t461,t462,t463,t465,t466,t467,t468,t469,t47,t470,t471,t472,t473,t474,t475,t476,t477,t478,t479,t480,t481,t482,t488,t491,t495,t496,t497,t498,t499,t5,t500,t501,t502,t503,t505,t507,t508,t509,t510,t511,t512,t513,t514,t516,t517,t520,t521,t522,t523,t524,t525,t526,t530,t531,t532,t533,t534,t535,t536,t537,t538,t539,t540,t542,t543,t545,t546,t547,t548,t550,t552,t553,t555,t556,t557,t559,t560,t561,t562,t564,t566,t568,t569,t570,t571,t572,t574,t576,t577,t578,t579,t580,t581,t584,t585,t586,t587,t588,t589,t59,t590,t592,t593,t594,t595,t596,t597,t598,t599,t6,t600,t604,t605,t607,t608,t609,t610,t611,t613,t614,t615,t616,t617,t618,t619,t62,t621,t622,t624,t626,t627,t629,t630,t636,t637,t638,t639,t640,t642,t645,t648,t653,t654,t655,t656,t659,t660,t661,t662,t663,t666,t667,t670,t671,t672,t673,t674,t675,t676,t678,t679,t681,t682,t683,t684,t685,t686,t687,t688,t689,t690,t691,t695,t697,t698,t7,t701,t702,t703,t704,t705,t706,t708,t709,t71,t712,t713,t714,t716,t717,t718,t719,t72,t720,t721,t722,t723,t725,t727,t73,t730,t732,t733,t736,t738,t74,t741,t743,t744,t745,t746,t747,t748,t749,t75,t750,t752,t753,t754,t755,t756,t757,t758,t759,t760,t761,t762,t763,t764,t765,t767,t768,t769,t77,t772,t773,t774,t775,t776,t777,t78,t780,t781,t782,t783,t787,t788,t789,t79,t790,t791,t792,t793,t797,t798,t799,t8,t80,t803,t804,t805,t812,t813,t814,t815,t816,t818,t819,t821,t822,t823,t824,t825,t828,t830,t831,t832,t833,t835,t836,t838,t839,t840,t841,t843,t844,t845,t846,t847,t848,t85,t851,t853,t854,t855,t856,t858,t861,t862,t863,t864,t869,t87,t871,t875,t876,t878,t88,t881,t882,t883,t886,t887,t888,t889,t89,t891,t893,t894,t895,t896,t897,t898,t899,t9,t90,t900,t901,t902,t903,t908,t909,t910,t911,t914,t916,t917,t918,t920,t921,t922,t923,t924,t925,t927,t928,t929,t930,t932,t933,t934,t935,t940,t941,t942,t943,t945,t946,t947,t948,t950,t951,t954,t956,t957,t958,t959,t96,t962,t970,t972,t973,t974,t975,t976,t977,t980,t982,t983,t984,t985,t986,t987,t988,t989,t990,t991,t992,t993,t994,t995,t998,t999});
end
function K = ft_2(ct)
dq1 = ct{1};
dq2 = ct{2};
dq3 = ct{3};
dq4 = ct{4};
dq5 = ct{5};
dq6 = ct{6};
t1000 = ct{7};
t1001 = ct{8};
t1004 = ct{9};
t1005 = ct{10};
t1006 = ct{11};
t1009 = ct{12};
t1010 = ct{13};
t1014 = ct{14};
t1015 = ct{15};
t1016 = ct{16};
t1018 = ct{17};
t1021 = ct{18};
t1022 = ct{19};
t1023 = ct{20};
t1024 = ct{21};
t1025 = ct{22};
t1026 = ct{23};
t1028 = ct{24};
t1029 = ct{25};
t1032 = ct{26};
t1033 = ct{27};
t1034 = ct{28};
t1036 = ct{29};
t1037 = ct{30};
t1039 = ct{31};
t1040 = ct{32};
t1041 = ct{33};
t1043 = ct{34};
t1044 = ct{35};
t1045 = ct{36};
t1046 = ct{37};
t1048 = ct{38};
t1049 = ct{39};
t1051 = ct{40};
t1053 = ct{41};
t1055 = ct{42};
t1056 = ct{43};
t1057 = ct{44};
t106 = ct{45};
t1060 = ct{46};
t1062 = ct{47};
t1066 = ct{48};
t1067 = ct{49};
t1068 = ct{50};
t1069 = ct{51};
t107 = ct{52};
t1070 = ct{53};
t1071 = ct{54};
t1072 = ct{55};
t1075 = ct{56};
t1076 = ct{57};
t1077 = ct{58};
t1078 = ct{59};
t108 = ct{60};
t1081 = ct{61};
t1083 = ct{62};
t1084 = ct{63};
t1089 = ct{64};
t1091 = ct{65};
t1093 = ct{66};
t1094 = ct{67};
t1095 = ct{68};
t1096 = ct{69};
t1097 = ct{70};
t1098 = ct{71};
t1100 = ct{72};
t1101 = ct{73};
t1104 = ct{74};
t1105 = ct{75};
t1109 = ct{76};
t1110 = ct{77};
t1111 = ct{78};
t1118 = ct{79};
t1119 = ct{80};
t1120 = ct{81};
t1121 = ct{82};
t1124 = ct{83};
t1126 = ct{84};
t1128 = ct{85};
t113 = ct{86};
t1131 = ct{87};
t1133 = ct{88};
t1138 = ct{89};
t1139 = ct{90};
t114 = ct{91};
t1146 = ct{92};
t1148 = ct{93};
t115 = ct{94};
t1151 = ct{95};
t1160 = ct{96};
t1166 = ct{97};
t1179 = ct{98};
t119 = ct{99};
t1195 = ct{100};
t120 = ct{101};
t1204 = ct{102};
t1205 = ct{103};
t121 = ct{104};
t1217 = ct{105};
t124 = ct{106};
t1268 = ct{107};
t1269 = ct{108};
t1270 = ct{109};
t130 = ct{110};
t132 = ct{111};
t133 = ct{112};
t135 = ct{113};
t136 = ct{114};
t138 = ct{115};
t14 = ct{116};
t140 = ct{117};
t141 = ct{118};
t144 = ct{119};
t146 = ct{120};
t15 = ct{121};
t150 = ct{122};
t151 = ct{123};
t152 = ct{124};
t154 = ct{125};
t156 = ct{126};
t158 = ct{127};
t159 = ct{128};
t16 = ct{129};
t160 = ct{130};
t161 = ct{131};
t162 = ct{132};
t163 = ct{133};
t164 = ct{134};
t166 = ct{135};
t167 = ct{136};
t168 = ct{137};
t169 = ct{138};
t17 = ct{139};
t170 = ct{140};
t171 = ct{141};
t172 = ct{142};
t175 = ct{143};
t177 = ct{144};
t178 = ct{145};
t179 = ct{146};
t18 = ct{147};
t180 = ct{148};
t181 = ct{149};
t184 = ct{150};
t185 = ct{151};
t186 = ct{152};
t187 = ct{153};
t188 = ct{154};
t189 = ct{155};
t19 = ct{156};
t190 = ct{157};
t191 = ct{158};
t192 = ct{159};
t194 = ct{160};
t196 = ct{161};
t197 = ct{162};
t198 = ct{163};
t199 = ct{164};
t2 = ct{165};
t20 = ct{166};
t200 = ct{167};
t202 = ct{168};
t203 = ct{169};
t204 = ct{170};
t209 = ct{171};
t21 = ct{172};
t210 = ct{173};
t211 = ct{174};
t212 = ct{175};
t213 = ct{176};
t214 = ct{177};
t215 = ct{178};
t217 = ct{179};
t218 = ct{180};
t219 = ct{181};
t22 = ct{182};
t220 = ct{183};
t221 = ct{184};
t222 = ct{185};
t225 = ct{186};
t227 = ct{187};
t228 = ct{188};
t23 = ct{189};
t232 = ct{190};
t233 = ct{191};
t234 = ct{192};
t235 = ct{193};
t236 = ct{194};
t238 = ct{195};
t239 = ct{196};
t241 = ct{197};
t242 = ct{198};
t244 = ct{199};
t245 = ct{200};
t246 = ct{201};
t248 = ct{202};
t251 = ct{203};
t255 = ct{204};
t256 = ct{205};
t257 = ct{206};
t258 = ct{207};
t26 = ct{208};
t260 = ct{209};
t261 = ct{210};
t262 = ct{211};
t263 = ct{212};
t264 = ct{213};
t265 = ct{214};
t266 = ct{215};
t267 = ct{216};
t268 = ct{217};
t27 = ct{218};
t273 = ct{219};
t274 = ct{220};
t278 = ct{221};
t282 = ct{222};
t283 = ct{223};
t287 = ct{224};
t288 = ct{225};
t289 = ct{226};
t291 = ct{227};
t292 = ct{228};
t293 = ct{229};
t294 = ct{230};
t295 = ct{231};
t296 = ct{232};
t298 = ct{233};
t3 = ct{234};
t30 = ct{235};
t300 = ct{236};
t301 = ct{237};
t302 = ct{238};
t303 = ct{239};
t304 = ct{240};
t305 = ct{241};
t307 = ct{242};
t310 = ct{243};
t313 = ct{244};
t315 = ct{245};
t316 = ct{246};
t319 = ct{247};
t321 = ct{248};
t322 = ct{249};
t323 = ct{250};
t326 = ct{251};
t327 = ct{252};
t328 = ct{253};
t329 = ct{254};
t330 = ct{255};
t331 = ct{256};
t332 = ct{257};
t333 = ct{258};
t334 = ct{259};
t336 = ct{260};
t337 = ct{261};
t340 = ct{262};
t341 = ct{263};
t343 = ct{264};
t344 = ct{265};
t345 = ct{266};
t346 = ct{267};
t347 = ct{268};
t348 = ct{269};
t349 = ct{270};
t35 = ct{271};
t351 = ct{272};
t353 = ct{273};
t354 = ct{274};
t355 = ct{275};
t356 = ct{276};
t357 = ct{277};
t358 = ct{278};
t361 = ct{279};
t362 = ct{280};
t364 = ct{281};
t365 = ct{282};
t366 = ct{283};
t367 = ct{284};
t368 = ct{285};
t373 = ct{286};
t374 = ct{287};
t377 = ct{288};
t379 = ct{289};
t38 = ct{290};
t380 = ct{291};
t381 = ct{292};
t382 = ct{293};
t384 = ct{294};
t386 = ct{295};
t387 = ct{296};
t388 = ct{297};
t389 = ct{298};
t392 = ct{299};
t393 = ct{300};
t395 = ct{301};
t396 = ct{302};
t397 = ct{303};
t398 = ct{304};
t399 = ct{305};
t4 = ct{306};
t403 = ct{307};
t404 = ct{308};
t405 = ct{309};
t406 = ct{310};
t407 = ct{311};
t408 = ct{312};
t409 = ct{313};
t41 = ct{314};
t410 = ct{315};
t411 = ct{316};
t414 = ct{317};
t415 = ct{318};
t416 = ct{319};
t417 = ct{320};
t42 = ct{321};
t420 = ct{322};
t421 = ct{323};
t424 = ct{324};
t425 = ct{325};
t426 = ct{326};
t427 = ct{327};
t428 = ct{328};
t429 = ct{329};
t43 = ct{330};
t431 = ct{331};
t434 = ct{332};
t435 = ct{333};
t436 = ct{334};
t437 = ct{335};
t438 = ct{336};
t439 = ct{337};
t443 = ct{338};
t444 = ct{339};
t448 = ct{340};
t449 = ct{341};
t45 = ct{342};
t450 = ct{343};
t451 = ct{344};
t452 = ct{345};
t453 = ct{346};
t454 = ct{347};
t455 = ct{348};
t456 = ct{349};
t457 = ct{350};
t460 = ct{351};
t461 = ct{352};
t462 = ct{353};
t463 = ct{354};
t465 = ct{355};
t466 = ct{356};
t467 = ct{357};
t468 = ct{358};
t469 = ct{359};
t47 = ct{360};
t470 = ct{361};
t471 = ct{362};
t472 = ct{363};
t473 = ct{364};
t474 = ct{365};
t475 = ct{366};
t476 = ct{367};
t477 = ct{368};
t478 = ct{369};
t479 = ct{370};
t480 = ct{371};
t481 = ct{372};
t482 = ct{373};
t488 = ct{374};
t491 = ct{375};
t495 = ct{376};
t496 = ct{377};
t497 = ct{378};
t498 = ct{379};
t499 = ct{380};
t5 = ct{381};
t500 = ct{382};
t501 = ct{383};
t502 = ct{384};
t503 = ct{385};
t505 = ct{386};
t507 = ct{387};
t508 = ct{388};
t509 = ct{389};
t510 = ct{390};
t511 = ct{391};
t512 = ct{392};
t513 = ct{393};
t514 = ct{394};
t516 = ct{395};
t517 = ct{396};
t520 = ct{397};
t521 = ct{398};
t522 = ct{399};
t523 = ct{400};
t524 = ct{401};
t525 = ct{402};
t526 = ct{403};
t530 = ct{404};
t531 = ct{405};
t532 = ct{406};
t533 = ct{407};
t534 = ct{408};
t535 = ct{409};
t536 = ct{410};
t537 = ct{411};
t538 = ct{412};
t539 = ct{413};
t540 = ct{414};
t542 = ct{415};
t543 = ct{416};
t545 = ct{417};
t546 = ct{418};
t547 = ct{419};
t548 = ct{420};
t550 = ct{421};
t552 = ct{422};
t553 = ct{423};
t555 = ct{424};
t556 = ct{425};
t557 = ct{426};
t559 = ct{427};
t560 = ct{428};
t561 = ct{429};
t562 = ct{430};
t564 = ct{431};
t566 = ct{432};
t568 = ct{433};
t569 = ct{434};
t570 = ct{435};
t571 = ct{436};
t572 = ct{437};
t574 = ct{438};
t576 = ct{439};
t577 = ct{440};
t578 = ct{441};
t579 = ct{442};
t580 = ct{443};
t581 = ct{444};
t584 = ct{445};
t585 = ct{446};
t586 = ct{447};
t587 = ct{448};
t588 = ct{449};
t589 = ct{450};
t59 = ct{451};
t590 = ct{452};
t592 = ct{453};
t593 = ct{454};
t594 = ct{455};
t595 = ct{456};
t596 = ct{457};
t597 = ct{458};
t598 = ct{459};
t599 = ct{460};
t6 = ct{461};
t600 = ct{462};
t604 = ct{463};
t605 = ct{464};
t607 = ct{465};
t608 = ct{466};
t609 = ct{467};
t610 = ct{468};
t611 = ct{469};
t613 = ct{470};
t614 = ct{471};
t615 = ct{472};
t616 = ct{473};
t617 = ct{474};
t618 = ct{475};
t619 = ct{476};
t62 = ct{477};
t621 = ct{478};
t622 = ct{479};
t624 = ct{480};
t626 = ct{481};
t627 = ct{482};
t629 = ct{483};
t630 = ct{484};
t636 = ct{485};
t637 = ct{486};
t638 = ct{487};
t639 = ct{488};
t640 = ct{489};
t642 = ct{490};
t645 = ct{491};
t648 = ct{492};
t653 = ct{493};
t654 = ct{494};
t655 = ct{495};
t656 = ct{496};
t659 = ct{497};
t660 = ct{498};
t661 = ct{499};
t662 = ct{500};
t663 = ct{501};
t666 = ct{502};
t667 = ct{503};
t670 = ct{504};
t671 = ct{505};
t672 = ct{506};
t673 = ct{507};
t674 = ct{508};
t675 = ct{509};
t676 = ct{510};
t678 = ct{511};
t679 = ct{512};
t681 = ct{513};
t682 = ct{514};
t683 = ct{515};
t684 = ct{516};
t685 = ct{517};
t686 = ct{518};
t687 = ct{519};
t688 = ct{520};
t689 = ct{521};
t690 = ct{522};
t691 = ct{523};
t695 = ct{524};
t697 = ct{525};
t698 = ct{526};
t7 = ct{527};
t701 = ct{528};
t702 = ct{529};
t703 = ct{530};
t704 = ct{531};
t705 = ct{532};
t706 = ct{533};
t708 = ct{534};
t709 = ct{535};
t71 = ct{536};
t712 = ct{537};
t713 = ct{538};
t714 = ct{539};
t716 = ct{540};
t717 = ct{541};
t718 = ct{542};
t719 = ct{543};
t72 = ct{544};
t720 = ct{545};
t721 = ct{546};
t722 = ct{547};
t723 = ct{548};
t725 = ct{549};
t727 = ct{550};
t73 = ct{551};
t730 = ct{552};
t732 = ct{553};
t733 = ct{554};
t736 = ct{555};
t738 = ct{556};
t74 = ct{557};
t741 = ct{558};
t743 = ct{559};
t744 = ct{560};
t745 = ct{561};
t746 = ct{562};
t747 = ct{563};
t748 = ct{564};
t749 = ct{565};
t75 = ct{566};
t750 = ct{567};
t752 = ct{568};
t753 = ct{569};
t754 = ct{570};
t755 = ct{571};
t756 = ct{572};
t757 = ct{573};
t758 = ct{574};
t759 = ct{575};
t760 = ct{576};
t761 = ct{577};
t762 = ct{578};
t763 = ct{579};
t764 = ct{580};
t765 = ct{581};
t767 = ct{582};
t768 = ct{583};
t769 = ct{584};
t77 = ct{585};
t772 = ct{586};
t773 = ct{587};
t774 = ct{588};
t775 = ct{589};
t776 = ct{590};
t777 = ct{591};
t78 = ct{592};
t780 = ct{593};
t781 = ct{594};
t782 = ct{595};
t783 = ct{596};
t787 = ct{597};
t788 = ct{598};
t789 = ct{599};
t79 = ct{600};
t790 = ct{601};
t791 = ct{602};
t792 = ct{603};
t793 = ct{604};
t797 = ct{605};
t798 = ct{606};
t799 = ct{607};
t8 = ct{608};
t80 = ct{609};
t803 = ct{610};
t804 = ct{611};
t805 = ct{612};
t812 = ct{613};
t813 = ct{614};
t814 = ct{615};
t815 = ct{616};
t816 = ct{617};
t818 = ct{618};
t819 = ct{619};
t821 = ct{620};
t822 = ct{621};
t823 = ct{622};
t824 = ct{623};
t825 = ct{624};
t828 = ct{625};
t830 = ct{626};
t831 = ct{627};
t832 = ct{628};
t833 = ct{629};
t835 = ct{630};
t836 = ct{631};
t838 = ct{632};
t839 = ct{633};
t840 = ct{634};
t841 = ct{635};
t843 = ct{636};
t844 = ct{637};
t845 = ct{638};
t846 = ct{639};
t847 = ct{640};
t848 = ct{641};
t85 = ct{642};
t851 = ct{643};
t853 = ct{644};
t854 = ct{645};
t855 = ct{646};
t856 = ct{647};
t858 = ct{648};
t861 = ct{649};
t862 = ct{650};
t863 = ct{651};
t864 = ct{652};
t869 = ct{653};
t87 = ct{654};
t871 = ct{655};
t875 = ct{656};
t876 = ct{657};
t878 = ct{658};
t88 = ct{659};
t881 = ct{660};
t882 = ct{661};
t883 = ct{662};
t886 = ct{663};
t887 = ct{664};
t888 = ct{665};
t889 = ct{666};
t89 = ct{667};
t891 = ct{668};
t893 = ct{669};
t894 = ct{670};
t895 = ct{671};
t896 = ct{672};
t897 = ct{673};
t898 = ct{674};
t899 = ct{675};
t9 = ct{676};
t90 = ct{677};
t900 = ct{678};
t901 = ct{679};
t902 = ct{680};
t903 = ct{681};
t908 = ct{682};
t909 = ct{683};
t910 = ct{684};
t911 = ct{685};
t914 = ct{686};
t916 = ct{687};
t917 = ct{688};
t918 = ct{689};
t920 = ct{690};
t921 = ct{691};
t922 = ct{692};
t923 = ct{693};
t924 = ct{694};
t925 = ct{695};
t927 = ct{696};
t928 = ct{697};
t929 = ct{698};
t930 = ct{699};
t932 = ct{700};
t933 = ct{701};
t934 = ct{702};
t935 = ct{703};
t940 = ct{704};
t941 = ct{705};
t942 = ct{706};
t943 = ct{707};
t945 = ct{708};
t946 = ct{709};
t947 = ct{710};
t948 = ct{711};
t950 = ct{712};
t951 = ct{713};
t954 = ct{714};
t956 = ct{715};
t957 = ct{716};
t958 = ct{717};
t959 = ct{718};
t96 = ct{719};
t962 = ct{720};
t970 = ct{721};
t972 = ct{722};
t973 = ct{723};
t974 = ct{724};
t975 = ct{725};
t976 = ct{726};
t977 = ct{727};
t980 = ct{728};
t982 = ct{729};
t983 = ct{730};
t984 = ct{731};
t985 = ct{732};
t986 = ct{733};
t987 = ct{734};
t988 = ct{735};
t989 = ct{736};
t990 = ct{737};
t991 = ct{738};
t992 = ct{739};
t993 = ct{740};
t994 = ct{741};
t995 = ct{742};
t998 = ct{743};
t999 = ct{744};
t996 = t8.*t974;
t997 = t8.*t975;
t1002 = -t987;
t1003 = -t988;
t1007 = t8.*t982;
t1008 = t8.*t983;
t1011 = -t998;
t1012 = -t999;
t1013 = -t1000;
t1017 = t5.*t986;
t1019 = t8.*t987;
t1020 = t8.*t988;
t1027 = -t1005;
t1030 = t8.*t992;
t1031 = -t1006;
t1035 = t8.*t999;
t1038 = -t1016;
t1042 = -t1028;
t1047 = -t1036;
t1050 = t8.*t1015;
t1052 = t8.*t1016;
t1054 = -t1037;
t1058 = t9.*t1023;
t1059 = t8.*t1024;
t1061 = t8.*t1006;
t1063 = -t1055;
t1064 = -t1056;
t1065 = -t1057;
t1073 = -t1069;
t1074 = -t1071;
t1079 = -t1075;
t1080 = -t1076;
t1082 = -t1077;
t1086 = -t1083;
t1087 = -t1084;
t1090 = -t1089;
t1102 = -t1096;
t1103 = t73.*7.67777073541389e-5;
t1106 = -t1104;
t1107 = -t1105;
t1108 = t5.*t7.*t30.*t72.*t74.*1.8197034170822e-22;
t1112 = t4.*t9.*t30.*t72.*t75.*1.530369361342075e-22;
t1113 = t5.*t7.*t9.*t30.*t72.*t74.*5.659386953851025e-22;
t1114 = t8.*t30.*t72.*t75.*3.356793907564468e-24;
t1115 = -t1110;
t1116 = t7.*t18.*t30.*t72.*t74.*3.719939515191737e-22;
t1122 = t7.*t9.*t30.*t72.*t74.*9.890501569818525e-23;
t1123 = t4.*t5.*t9.*t30.*t72.*t75.*3.128466653771177e-22;
t1125 = -t1118;
t1127 = -t1120;
t1129 = t4.*t5.*t8.*t30.*t72.*t74.*3.060738722684151e-22;
t1130 = t4.*t18.*t30.*t72.*t75.*4.759540657477059e-22;
t1135 = -t1126;
t1136 = t9.*t30.*t72.*t74.*6.005538711575609e-29;
t1137 = t4.*t5.*t30.*t72.*t75.*8.317905230417136e-23;
t1140 = -t1133;
t1141 = t5.*t7.*t17.*t30.*t72.*t74.*(-1.8197034170822e-22);
t1142 = t4.*t5.*t8.*t9.*t30.*t72.*t74.*4.759540657477059e-22;
t1143 = t4.*t8.*t18.*t30.*t72.*t74.*3.128466653771177e-22;
t1144 = t4.*t8.*t9.*t30.*t72.*t74.*1.663581046083427e-22;
t1147 = t4.*t30.*t72.*t75.*2.374951658244784e-22;
t1149 = t7.*t17.*t18.*t30.*t72.*t74.*1.859969757595868e-22;
t1150 = t5.*t8.*t30.*t72.*t75.*6.005538711575609e-29;
t1152 = t5.*t7.*t9.*t17.*t30.*t72.*t74.*2.829693476925513e-22;
t1155 = t5.*t30.*t72.*t74.*7.875493318833269e-29;
t1156 = -t1148;
t1161 = t7.*t30.*t72.*t74.*4.499077832247571e-22;
t1167 = t7.*t9.*t17.*t30.*t72.*t74.*(-9.890501569818525e-23);
t1169 = t4.*t8.*t30.*t72.*t74.*1.126529406341455e-22;
t1170 = -t1160;
t1173 = t9.*t17.*t30.*t72.*t74.*1.201107742315122e-28;
t1174 = -t1166;
t1175 = t8.*t9.*t30.*t72.*t75.*7.875493318833269e-29;
t1177 = t4.*t7.*t8.*t9.*t30.*t72.*t74.*7.140955373864693e-29;
t1178 = t5.*t17.*t30.*t72.*t74.*1.575098663766654e-28;
t1180 = t7.*t17.*t30.*t72.*t74.*6.697564202296239e-23;
t1182 = t4.*t5.*t7.*t8.*t30.*t72.*t74.*9.364446561398189e-29;
t1188 = t17.*t30.*t72.*t74.*2.783302668250669e-22;
t1190 = t4.*t7.*t8.*t30.*t72.*t74.*1.654759139894217e-22;
t1192 = t9.*t30.*t72.*t75.*1.463238712860231e-21;
t1194 = t5.*t30.*t72.*t75.*7.953034901571333e-22;
t1196 = t5.*t8.*t30.*t72.*t74.*1.463238712860231e-21;
t1197 = t8.*t9.*t30.*t72.*t74.*7.953034901571333e-22;
t1198 = t30.*t72.*t75.*6.180449594294637e-22;
t1199 = t8.*t30.*t72.*t74.*1.154708176178584e-21;
t1200 = t30.*t72.*t74.*1.406496925043394e-22;
t1201 = t4.*t30.*t72.*t74.*1.485300862305337e-21;
t81 = -t79;
t216 = t4.*t9.*t191;
t243 = t4.*t5.*t198;
t250 = -t236;
t252 = -t238;
t254 = -t242;
t259 = -t245;
t279 = -t264;
t299 = -t283;
t314 = -t300;
t339 = -t330;
t342 = -t334;
t359 = -t358;
t375 = t22.*t367;
t376 = t23.*t367;
t506 = -t477;
t573 = t5.*t566;
t575 = t9.*t566;
t582 = t5.*t576;
t583 = t9.*t576;
t602 = -t594;
t606 = -t597;
t620 = -t611;
t623 = -t613;
t625 = -t616;
t628 = t17.*t594;
t631 = -t621;
t635 = -t630;
t641 = t16.*t17.*t586;
t643 = t16.*t17.*t587;
t644 = -t636;
t649 = t477./8.112963841460668e+31;
t650 = t17.*t621;
t652 = -t645;
t664 = -t661;
t665 = -t663;
t669 = -t667;
t770 = -t764;
t771 = -t765;
t778 = t8.*t764;
t795 = -t776;
t796 = t8.*t769;
t802 = -t783;
t808 = t22.*t744;
t809 = t22.*t745;
t810 = t23.*t744;
t811 = t23.*t745;
t817 = -t792;
t829 = t8.*t783;
t834 = t22.*t759;
t837 = t23.*t759;
t842 = -t821;
t852 = t8.*t781;
t860 = -t838;
t865 = t8.*t816;
t866 = t5.*t818;
t867 = t8.*t821;
t868 = -t840;
t870 = -t846;
t877 = t8.*t831;
t879 = t8.*t832;
t890 = t8.*t843;
t892 = t8.*t844;
t905 = t8.*t862;
t906 = t9.*t861;
t907 = t8.*t863;
t913 = -t900;
t915 = -t910;
t931 = -t928;
t936 = -t933;
t937 = -t934;
t938 = -t935;
t939 = t185+t340;
t949 = -t940;
t952 = t74+t538;
t960 = -t954;
t961 = t948.^2;
t963 = -t957;
t964 = t5.*t948;
t965 = t9.*t948;
t966 = -t962;
t1117 = -t1112;
t1132 = -t1123;
t1134 = t17.*t1108;
t1145 = -t1136;
t1153 = -t1147;
t1154 = t17.*t1122;
t1157 = -t1149;
t1158 = -t1150;
t1159 = t41.*t948;
t1162 = t42.*t948;
t1163 = t43.*t948;
t1164 = -t1152;
t1165 = t45.*t948;
t1168 = -t1155;
t1171 = -t1161;
t1176 = -t1169;
t1181 = t59.*t948;
t1186 = t62.*t948;
t1189 = -t1188;
t1191 = -t1190;
t1193 = -t1192;
t1202 = -t1201;
t1245 = t192+t566+t671;
t1246 = t189+t190+t361+t373;
t1271 = t197+t204+t564+t576+t678;
t1272 = t194+t202+t569+t574+t676;
t1273 = t948.*t1270;
t378 = -t376;
t657 = -t649;
t859 = -t811;
t884 = -t837;
t955 = t939.^2;
t968 = t4.*t952;
t969 = t8.*t952;
t971 = -t965;
t1085 = t188+t375;
t1184 = t964.*(-3.146556677756745e-13);
t1215 = t810+t834;
t1216 = t809+t837;
t1224 = -t3.*(t811-t834);
t1226 = -t7.*(t811-t834);
t1249 = t339+t377+t381+t382;
t1260 = -t4.*(t7.*(t811-t834)+(t3.*t30.*t72.*(t26-t27))./8.112963841460668e+31);
t1261 = -t8.*(t7.*(t811-t834)+(t3.*t30.*t72.*(t26-t27))./8.112963841460668e+31);
t1266 = t4.*(t7.*(t811-t834)+(t3.*t30.*t72.*(t26-t27))./8.112963841460668e+31);
t1280 = t77+t540+t1272;
t1342 = t80+t203+t210+t221+t552+t561+t575+t577+t582+t683+t685;
t1343 = t81+t209+t211+t222+t553+t557+t578+t580+t583+t679+t686;
t1434 = t199+t212+t214+t215+t220+t225+t235+t252+t254+t263+t274+t301+t310+t387+t395+t398+t408+t416+t421+t434+t452+t455+t456+t466+t468+t472+t479+t497+t502+t510+t517+t535+t537+t543+t545+t556+t559+t684+t688+t689+t690+t695+t702+t705+t706+t708+t712+t717+t718+t721+t725+t748+t752+t753+t756+t762+t767+t797+t804+t824+t836+t848+t853+t866+t875+t878+t881+t883+t891+t894+t896+t899+t906+t914+t916+t921+t941+t943+t946+t950+t956+t958+t991+t1017+t1026+t1029+t1049+t1051+t1058+t1068+t1070+t1093+t1097+t1100;
t1435 = t213+t228+t239+t243+t244+t250+t256+t259+t265+t266+t279+t293+t299+t304+t313+t314+t323+t359+t393+t403+t411+t415+t420+t426+t437+t439+t454+t461+t463+t465+t471+t474+t478+t491+t496+t499+t501+t509+t516+t548+t550+t562+t681+t691+t698+t703+t709+t716+t719+t720+t723+t727+t733+t736+t741+t743+t746+t747+t749+t750+t755+t760+t761+t768+t770+t773+t774+t790+t791+t793+t796+t802+t815+t830+t832+t842+t844+t852+t863+t865+t877+t882+t886+t890+t898+t905+t908+t911+t917+t920+t922+t924+t949+t960+t963+t984+t989+t992+t994+t1002+t1010+t1015+t1024+t1027+t1033+t1040+t1043+t1045+t1046+t1053+t1062+t1063+t1066+t1073+t1074+t1079+t1094+t1098+t1101;
et1 = t218+t232+t234+t246+t248+t251+t257+t258+t260+t261+t267+t268+t278+t282+t287+t289+t291+t292+t294+t295+t296+t298+t303+t305+t307+t315+t316+t319+t321+t322+t326+t327+t328+t329+t331+t332+t336+t337+t341+t343+t344+t345+t346+t347+t348+t349+t351+t353+t354+t365+t366+t374+t389+t404+t409+t414+t428+t431+t435+t436+t438+t444+t448+t451+t453+t462+t469+t470+t475+t476+t480+t482+t488+t495+t500+t505+t507+t508+t511+t520+t522+t524+t536+t542+t546+t547+t555+t560+t579+t584+t586+t587+t589+t592+t595+t596+t598+t599+t600+t602+t604+t607+t608+t609+t610+t614+t615+t618+t619+t620+t622+t623+t624+t625+t626+t627+t628+t629+t631+t635+t637+t638+t639+t640+t641+t642+t643+t644+t650+t652+t653+t654+t656+t659+t660+t664+t665+t666+t669+t675+t682+t701+t757+t758+t763+t771+t772+t777+t780+t782+t795+t799+t805+t813+t814+t817+t819+t822+t825+t833+t839+t851+t855+t858+t860+t864+t868+t870+t871+t876+t887+t889+t893+t895+t897+t901+t902+t903+t909+t913+t915+t918+t923+t932+t938+t942+t945+t947+t951+t959+t966+t970+t972+t976+t977+t980+t990+t993+t1001+t1004;
et2 = t1011+t1013+t1014+t1021+t1025+t1034+t1041+t1042+t1044+t1047+t1048+t1060+t1064+t1065+t1067+t1072+t1080+t1081+t1090+t1095+t1102+t1103+t1106+t1107+t1108+t1109+t1111+t1113+t1114+t1115+t1116+t1117+t1119+t1121+t1122+t1124+t1125+t1127+t1129+t1130+t1132+t1135+t1137+t1139+t1140+t1141+t1142+t1143+t1144+t1145+t1151+t1153+t1156+t1157+t1158+t1164+t1167+t1168+t1170+t1171+t1173+t1175+t1176+t1177+t1178+t1179+t1180+t1182+t1189+t1191+t1193+t1194+t1196+t1197+t1198+t1199+t1200+t1202;
et3 = 3.626861556360138e-4;
t1436 = et1+et2+et3;
t1088 = t187+t378;
t1092 = t3.*t1085;
t1172 = t968.*4.20092050615074e-6;
t1183 = t968.*3.146556677756745e-13;
t1187 = t968.*4.126305279697715e-13;
t1203 = t955.*4.040985049072001e-70;
t1206 = t532+t968;
t1207 = t539+t969;
t1209 = -t5.*(t531-t969);
t1210 = -t9.*(t531-t969);
t1218 = t834+t859;
t1219 = t808+t884;
t1220 = t3.*t1216;
t1221 = t4.*t1215;
t1222 = t7.*t1216;
t1223 = t8.*t1215;
t1232 = t5.*(t531-t969).*(-1.744166498897461e-6);
t1233 = -t42.*(t531-t969);
t1234 = -t43.*(t531-t969);
t1235 = t9.*(t531-t969).*(-3.383302988283333e-6);
t1236 = t5.*(t531-t969).*1.744166498897461e-6;
t1237 = t5.*(t531-t969).*1.246862701090643e-6;
t1239 = t9.*(t531-t969).*(-3.146556677756745e-13);
t1241 = t9.*(t531-t969).*3.146556677756745e-13;
t1243 = t5.*(t531-t969).*(-4.126305279697715e-13);
t1244 = t5.*(t531-t969).*4.126305279697715e-13;
t1252 = t655+t1226;
t1256 = t662+t1224;
t1285 = -t1268.*(t531-t969);
t1326 = -t1246.*(t965+t5.*(t531-t969));
t1334 = t1246.*(t965+t5.*(t531-t969)).*(-7.26735e-3);
t1335 = t1246.*(t965+t5.*(t531-t969)).*7.26735e-3;
t1336 = t1246.*(t965+t5.*(t531-t969)).*(-7.26350610236655e-5);
t1338 = t1246.*(t965+t5.*(t531-t969)).*(-1.40259855e-11);
t1339 = t1246.*(t965+t5.*(t531-t969)).*1.40259855e-11;
t1099 = t3.*t1088;
t1185 = -t1183;
t1208 = t1206.^2;
t1211 = t506+t1092;
t1212 = (t477-t1092).^2;
t1225 = t4.*t1219;
t1227 = t8.*t1219;
t1250 = t648+t1222;
t1251 = t657+t1220;
t1255 = (t649-t1220).^2;
t1257 = -t5.*(t649-t1220);
t1258 = -t9.*(t649-t1220);
t1262 = t1256.^2;
t1263 = t964+t1210;
t1264 = t5.*t1256;
t1265 = t9.*t1256;
t1267 = t971+t1209;
t1274 = t1206.*t1246;
t1282 = -t1206.*(t965+t5.*(t531-t969));
t1283 = t1206.*(t965+t5.*(t531-t969));
t1284 = t1206.*t1269;
t1414 = t198+t333+t384+t424+t514+t521+t534+t687+t754+t787+t828+t841+t861+t927+t930+t937+t1023+t1082+t1087+t1159+t1162+t1187+t1234+t1236;
t1417 = t227+t241+t386+t396+t406+t425+t443+t467+t670+t697+t704+t713+t732+t816+t835+t862+t869+t888+t907+t1003+t1031+t1039+t1059+t1172+t1184+t1186+t1241+t1244;
t1213 = t512+t1099;
t1228 = t1208.*1.33637579258949e-4;
t1229 = t1208.*7.26350610236655e-5;
t1230 = t1208.*4.20092050615074e-6;
t1238 = t1208.*3.146556677756745e-13;
t1242 = t1208.*4.126305279697715e-13;
t1247 = t1212.*4.040985049072001e-70;
t1253 = t4.*t1250;
t1254 = t8.*t1250;
t1275 = -t1274;
t1276 = t1274.*1.33637579258949e-4;
t1277 = t1274.*7.26735e-3;
t1278 = t1274.*7.26350610236655e-5;
t1281 = t1206.*t1263;
t1292 = t1225+t1261;
t1294 = t1227+t1266;
t1299 = t1283.*(-7.26350610236655e-5);
t1301 = t1283.*7.26350610236655e-5;
t1302 = t1283.*(-1.246862701090643e-6);
t1304 = t1283.*(-1.744166498897461e-6);
t1305 = t1283.*1.246862701090643e-6;
t1306 = t1283.*1.744166498897461e-6;
t1310 = t1283.*(-1.40259855e-11);
t1311 = t1283.*(-4.126305279697715e-13);
t1312 = t1283.*1.40259855e-11;
t1313 = t1283.*4.126305279697715e-13;
t1325 = t1246.*t1263;
t1341 = t961+t1255+t1262;
t1413 = t191+t342+t379+t399+t513+t525+t533+t673+t730+t789+t812+t818+t823+t929+t931+t936+t986+t1078+t1086+t1163+t1165+t1185+t1235+t1237;
t1214 = t1213.^2;
t1231 = -t1229;
t1240 = -t1238;
t1259 = -t1253;
t1279 = -t1278;
t1286 = t1221+t1254;
t1291 = t1281.*1.33637579258949e-4;
t1295 = t1281.*1.246862701090643e-6;
t1296 = t1281.*3.383302988283333e-6;
t1297 = t5.*t1292;
t1298 = t9.*t1292;
t1300 = t1294.^2;
t1307 = t1281.*3.146556677756745e-13;
t1308 = t1281.*1.40259855e-11;
t1327 = -t1325;
t1331 = t1325.*1.33637579258949e-4;
t1332 = t1325.*7.26735e-3;
t1337 = t1325.*1.40259855e-11;
t1349 = t1249.*t1294.*(t26-t27).*(-7.596454196607839e-68);
t1355 = t1249.*t1294.*(t26-t27).*(-1.015171749786156e-71);
t1356 = t1249.*t1294.*(t26-t27).*(-5.520609140571798e-70);
t1357 = t1249.*t1294.*(t26-t27).*(-5.517689141340903e-72);
t1358 = t1249.*t1294.*(t26-t27).*1.015171749786156e-71;
t1359 = t1249.*t1294.*(t26-t27).*5.520609140571798e-70;
t1248 = t1214.*4.040985049072001e-70;
t1287 = t1223+t1259;
t1288 = t5.*t1286;
t1289 = t9.*t1286;
t1303 = -t1298;
t1309 = -t1307;
t1318 = t1300.*1.33637579258949e-4;
t1319 = t1300.*7.26350610236655e-5;
t1321 = t1300.*4.20092050615074e-6;
t1328 = t1300.*3.146556677756745e-13;
t1330 = t1300.*4.126305279697715e-13;
t1333 = -t1331;
t1346 = t1265+t1297;
t1290 = t1287.^2;
t1293 = -t1289;
t1320 = -t1319;
t1329 = -t1328;
t1340 = t1203+t1247+t1248;
t1344 = t1258+t1288;
t1347 = t1264+t1303;
t1348 = (t47.*t1249.*t1287)./1.316403645856965e+67;
t1350 = t47.*t1249.*t1287.*1.015171749786156e-71;
t1351 = t47.*t1249.*t1287.*5.520609140571798e-70;
t1352 = t47.*t1249.*t1287.*5.517689141340903e-72;
t1361 = t47.*t1249.*(t1289+t5.*(t649-t1220)).*(-7.596454196607839e-68);
t1362 = t1249.*t1346.*(t26-t27).*(-7.596454196607839e-68);
t1367 = t47.*t1249.*(t1289+t5.*(t649-t1220)).*(-1.015171749786156e-71);
t1368 = t47.*t1249.*(t1289+t5.*(t649-t1220)).*(-5.520609140571798e-70);
t1369 = t47.*t1249.*(t1289+t5.*(t649-t1220)).*5.520609140571798e-70;
t1372 = t1249.*t1346.*(t26-t27).*(-5.520609140571798e-70);
t1373 = t47.*t1249.*(t1289+t5.*(t649-t1220)).*(-1.065477564130357e-78);
t1374 = t1249.*t1346.*(t26-t27).*(-5.517689141340903e-72);
t1375 = t1249.*t1346.*(t26-t27).*5.520609140571798e-70;
t1376 = t47.*t1249.*(t1289+t5.*(t649-t1220)).*1.065477564130357e-78;
t1380 = t1249.*t1346.*(t26-t27).*(-1.065477564130357e-78);
t1381 = t1249.*t1346.*(t26-t27).*1.065477564130357e-78;
t1386 = -t1287.*(t1289+t5.*(t649-t1220));
t1387 = t1294.*t1346;
t1390 = t1287.*(t1289+t5.*(t649-t1220)).*(-1.33637579258949e-4);
t1393 = t1287.*(t1289+t5.*(t649-t1220)).*(-1.246862701090643e-6);
t1394 = t1287.*(t1289+t5.*(t649-t1220)).*(-3.383302988283333e-6);
t1397 = t1287.*(t1289+t5.*(t649-t1220)).*(-3.146556677756745e-13);
t1398 = t1287.*(t1289+t5.*(t649-t1220)).*(-1.40259855e-11);
t1399 = t1287.*(t1289+t5.*(t649-t1220)).*3.146556677756745e-13;
t1314 = t1290.*1.33637579258949e-4;
t1315 = t1290.*7.26350610236655e-5;
t1317 = t1290.*4.20092050615074e-6;
t1322 = t1290.*3.146556677756745e-13;
t1324 = t1290.*4.126305279697715e-13;
t1345 = t1257+t1293;
t1353 = -t1350;
t1354 = -t1351;
t1360 = (t47.*t1249.*t1344)./1.316403645856965e+67;
t1363 = t1249.*t1347.*(t26-t27).*(-7.596454196607839e-68);
t1364 = t47.*t1249.*t1344.*5.520609140571798e-70;
t1365 = t47.*t1249.*t1344.*5.517689141340903e-72;
t1370 = t47.*t1249.*t1344.*1.065477564130357e-78;
t1377 = t1249.*t1347.*(t26-t27).*(-1.015171749786156e-71);
t1378 = t1249.*t1347.*(t26-t27).*(-5.520609140571798e-70);
t1379 = t1249.*t1347.*(t26-t27).*5.520609140571798e-70;
t1382 = t1249.*t1347.*(t26-t27).*(-1.065477564130357e-78);
t1383 = t1249.*t1347.*(t26-t27).*1.065477564130357e-78;
t1384 = t1208+t1290+t1300;
t1385 = t1287.*t1344;
t1388 = t1294.*t1347;
t1400 = t1387.*7.26350610236655e-5;
t1402 = t1387.*1.744166498897461e-6;
t1403 = t1387.*1.246862701090643e-6;
t1406 = t1387.*1.40259855e-11;
t1407 = t1387.*4.126305279697715e-13;
t1411 = t1275+t1348+t1349;
t1316 = -t1315;
t1323 = -t1322;
t1366 = -t1364;
t1371 = -t1370;
t1389 = t1385.*7.26350610236655e-5;
t1391 = t1385.*1.744166498897461e-6;
t1392 = t1385.*1.246862701090643e-6;
t1395 = t1385.*1.40259855e-11;
t1396 = t1385.*4.126305279697715e-13;
t1401 = t1388.*1.33637579258949e-4;
t1404 = t1388.*1.246862701090643e-6;
t1405 = t1388.*3.383302988283333e-6;
t1408 = t1388.*3.146556677756745e-13;
t1409 = t1388.*1.40259855e-11;
t1412 = t85+t87+t107+t113+t114+t140+t1277+t1354+t1359;
t1415 = t1326+t1360+t1362;
t1416 = t1327+t1361+t1363;
t1418 = t78+t88+t158+t170+t178+t1332+t1369+t1379;
t1420 = t1281+t1386+t1388;
t1421 = t1283+t1385+t1387;
t1425 = t108+t132+t136+t138+t146+t152+t160+t167+t1279+t1337+t1352+t1357+t1376+t1383;
t1428 = t96+t133+t156+t166+t168+t172+t175+t177+t1333+t1336+t1365+t1367+t1374+t1377;
et4 = t90+t119+t150+t161-t168+t169-t172-t177+t1331-t1365+t1246.*(t965+t5.*(t531-t969)).*7.26350610236655e-5+t47.*t1249.*(t1289+t5.*(t649-t1220)).*1.015171749786156e-71;
et5 = t1249.*t1346.*(t26-t27).*5.517689141340903e-72;
et6 = t1249.*t1347.*(t26-t27).*1.015171749786156e-71;
t1429 = -t1206.*(et4+et5+et6);
t1410 = -t1408;
t1419 = t89+t106+t159+t164+t179+t1335+t1366+t1375;
t1422 = t1228+t1312+t1314+t1318+t1395+t1406;
t1423 = t1231+t1308+t1316+t1320+t1398+t1409;
t1424 = t115+t120+t124+t130+t135+t144+t151+t162+t1276+t1339+t1353+t1358+t1371+t1381;
t1427 = -t1425.*(t965+t5.*(t531-t969));
t1430 = t1291+t1301+t1389+t1390+t1400+t1401;
t1431 = t1240+t1296+t1305+t1323+t1329+t1392+t1394+t1403+t1405;
t1432 = t1242+t1295+t1306+t1324+t1330+t1391+t1393+t1402+t1404;
t1426 = t1263.*t1424;
t1433 = t1230+t1309+t1313+t1317+t1321+t1396+t1399+t1407+t1410;
et7 = t5.*1.603650951107388e-6+t9.*8.71620732283986e-7+t17.*5.902365793397849e-7-t20.*7.291452122456316e-7;
et8 = t5.*t17.*(-1.603650951107388e-6)-t9.*t17.*8.71620732283986e-7-t17.*t18.*1.639136489385872e-6+t4.*t5.*t8.*8.252610559395431e-13;
et9 = t4.*t8.*t9.*6.293113355513489e-13-t5.*t9.*t17.*2.493725402181286e-6+9.148624944245897e-6;
et10 = t5.*8.195215631096216e-7+t7.*6.334299027523179e-7;
et11 = t9.*4.454285918434201e-7+t17.*3.016314764575132e-7+t141+t154+t163+t171+t180+t184+t233+t255+t262+t273+t288+t302+t362;
et12 = t3.*t4.*1.069583140309415e-6-t5.*t7.*3.546806877605634e-13;
et13 = t7.*t9.*(-2.7046541903611e-13)-t5.*t17.*8.195215631096216e-7;
et14 = t7.*t17.*(-1.253488085959302e-6)-t9.*t17.*4.454285918434201e-7;
et15 = t17.*t18.*(-8.376559107229145e-7)+t4.*t5.*t8.*4.217371804444381e-13;
et16 = t4.*t7.*t8.*(-5.073437414621283e-7)+t4.*t8.*t9.*3.216000396080637e-13;
et17 = t3.*t4.*t18.*(-2.143506553146841e-6)+t5.*t7.*t17.*7.093613755211269e-13;
et18 = t5.*t9.*t17.*(-1.274380648825446e-6)+t7.*t9.*t17.*5.4093083807222e-13;
et19 = t3.*t4.*t5.*t9.*1.408936125616489e-6+t4.*t5.*t7.*t8.*1.378434177095879e-6;
et20 = t4.*t7.*t8.*t9.*7.492102979241942e-7+t4.*t7.*t8.*t18.*1.408936125616489e-6;
et21 = t4.*t5.*t7.*t8.*t9.*2.143506553146841e-6+4.675266403474358e-6;
et22 = (dq1.*t1435)./2.0+(dq2.*(t213+t228+t239+t243+t244+t250+t256+t259+t265+t266+t279+t293+t299+t304+t313+t314+t323+t359+t393+t411+t420+t426+t463+t465+t478+t550+t681+t691+t698+t703+t709+t716+t719+t720+t723+t727+t733+t736+t741+t743+t746+t747+t749+t750+t755+t760+t761+t768+t773+t774+t791+t793+t830+t842+t863+t865+t905+t908+t917+t920+t922+t924+t963+t1002+t1024+t1040+t1043+t1066+t1074+t1079+t1101))./2.0+(dq6.*(t8.*t1433-t4.*t9.*(-t1238+t1296+t1305+t1323+t1329+t1392+t1394+t1403+t1405)+t8.*t9.*(t1229-t1308+t1315+t1319-t1409+t1287.*(t1289+t5.*(t649-t1220)).*1.40259855e-11).*(3.0./5.0e+2)+t5.*t8.*t1422.*(3.0./5.0e+2)+t4.*t5.*t1432))./2.0;
et23 = (dq5.*(t181-t8.*t186+t4.*t5.*t368-t4.*t9.*t364))./2.0+(dq4.*(et7+et8+et9))./2.0+(dq3.*(et10+et11+et12+et13+et14+et15+et16+et17+et18+et19+et20+et21))./2.0;
et24 = t218+t232+t234+t246+t248+t251+t257+t258+t260+t261+t267+t268+t278+t282+t287+t289+t291+t292+t294+t295+t296+t298+t303+t305+t307+t315+t316+t319+t321+t322+t326+t327+t328+t329+t331+t332+t336+t337+t341+t343+t344+t345+t346+t347+t348+t349+t351+t353+t354+t365+t366+t374+t404+t444+t451+t453+t476+t488+t505+t507+t520+t524+t546+t555+t579+t584+t586+t587+t589+t592+t596+t599+t600+t602+t604+t607+t608+t609+t610+t614+t615+t618+t619+t620+t622+t623+t624+t625+t626+t627+t628+t629+t631+t635+t637+t638+t639+t640+t641+t642+t643+t644+t650+t652+t653+t654+t656+t659+t660+t664+t665+t666+t669+t675+t682+t701+t757+t758+t763+t772+t777+t782+t795+t813+t822+t825+t839+t858+t860+t864+t870+t871+t893+t903+t913+t918+t923+t932+t938+t947+t966+t970+t972+t976+t980+t1001+t1021+t1034+t1041+t1072+t1090+t1103+t1106+t1107+t1108+t1109+t1111+t1113+t1114+t1115+t1116+t1117+t1119+t1121+t1122+t1124+t1125+t1127+t1129+t1130+t1132+t1135+t1137+t1139+t1140+t1141+t1142+t1143+t1144+t1145+t1151+t1153+t1156+t1157+t1158+t1164+t1167+t1168+t1170+t1171+t1173+t1175+t1176+t1177+t1178+t1179+t1180+t1182+t1189+t1191;
et25 = t1193+t1194+t1196+t1197+t1198+t1199+t1200+t1202+3.626861556360138e-4;
et26 = t7.*4.434404699592312e-7;
et27 = t74.*1.343796452840321e-8;
et28 = t75.*8.307571936196077e-6+t393+t738.*(t965+t5.*(t531-t969));
et29 = t1342.*(t8.*7.26350610236655e-5+t4.*t9.*1.40259855e-11+t8.*t9.*4.36041e-5);
et30 = t30.*t72.*3.910962551211394e-22+t181.*t948+t4.*t1272.*7.051078772420001e-7+t8.*t1271.*7.051078772420001e-7-t714.*t1263+t1091.*t1206;
et31 = (t4.*2.257319918256733e-6-t8.*7.291452964015446e-7).*(t531-t969);
et32 = -t1343.*(t8.*1.33637579258949e-4+t4.*t5.*1.40259855e-11+t5.*t8.*4.36041e-5);
et33 = -t1206.*(t4.*7.291452964015446e-7-t8.*5.878412210495409e-7)+t1280.*(t4.*t5.*7.26350610236655e-5-t4.*t9.*1.33637579258949e-4);
et34 = -t1245.*(t4.*1.35652529206996e-4-t8.*6.185538795558e-5);
et35 = t3.*t30.*t72.*1.291537098619388e-21;
et36 = t7.*t30.*t72.*(-1.670883952997876e-24);
et37 = t955.*3.835762748795343e-73;
et38 = t1212.*3.835762748795343e-73;
et39 = t1214.*3.835762748795343e-73;
et40 = t955.*2.672078334207073e-72;
et41 = t1212.*2.672078334207073e-72;
et42 = t1214.*2.672078334207073e-72;
et43 = t955.*2.060956449549905e-68;
et44 = t1212.*2.060956449549905e-68;
et45 = t1214.*2.060956449549905e-68;
et46 = t955.*9.397632428359433e-69;
et47 = t1212.*9.397632428359433e-69;
et48 = t1214.*9.397632428359433e-69;
et49 = t368.*(t965+t5.*(t531-t969))-t5.*t1342.*1.40259855e-11-t9.*t1343.*1.40259855e-11-t186.*t1206+t364.*t1263+t355.*t1280+t948.*t1340+(t531-t8.*t74+t8.*t530).*(et37+et38+et39);
et50 = (et40+et41+et42).*(t532+t4.*t74-t4.*t7.*t30.*t72.*5.673626844500105e-17)+t1271.*(et43+et44+et45)+t1272.*(et46+et47+et48);
et51 = (dq1.*t1436)./2.0-(dq3.*(-t380+t427-t581-t588+t617-t973+t1022-t1131+t1146+t1195+t1273-t1284+t1426+t1427+t1429-t1217.*t1245+t1204.*t1272+t1205.*t1271+t1280.*t1412-t1342.*t1419+t1343.*t1418+t1268.*(t531-t969)))./2.0+(dq2.*(et24+et25))./2.0+(dq4.*(et26+et27+et28+et29+et30+et31+et32+et33+et34+et35+et36))./2.0;
et52 = (dq6.*(t1432.*(t965+t5.*(t531-t969))+t1206.*t1433+t1280.*t1430-t1343.*t1422+t1263.*(-t1238+t1296+t1305+t1323+t1329+t1392+t1394+t1403+t1405)+t1342.*(t1229-t1308+t1315+t1319-t1409+t1287.*(t1289+t5.*(t649-t1220)).*1.40259855e-11)))./2.0+(dq5.*(et49+et50))./2.0;
et53 = t1281.*8.01825475553694e-7+t1283.*4.35810366141993e-7+t1385.*4.35810366141993e-7+t1387.*4.35810366141993e-7;
et54 = t1388.*8.01825475553694e-7-t1287.*(t1289+t5.*(t649-t1220)).*8.01825475553694e-7+t9.*t1432+t5.*(-t1238+t1296+t1305+t1323+t1329+t1392+t1394+t1403+t1405);
et55 = t955./6.582018229284824e+63+t1212./6.582018229284824e+63;
et56 = t1214./6.582018229284824e+63;
et57 = t1274.*4.36041e-5+t3.*t5.*6.892170885479394e-7-t4.*t5.*2.227142959217101e-7;
et58 = t3.*t9.*3.746051489620971e-7+t4.*t9.*4.097607815548108e-7+t5.*t1424-t9.*t1425+t1270.*t1341;
et59 = t5.*t7.*t8.*3.746051489620971e-7-t7.*t8.*t9.*6.892170885479394e-7;
et60 = t47.*t1249.*t1287.*(-3.312365484343079e-72);
et61 = t1249.*t1294.*(t26-t27).*3.312365484343079e-72;
et62 = t4.*(-2.117495204325297e-7);
et63 = t8.*9.655440125097679e-8+t75.*2.659783725725934e-6+t689;
et64 = t968.*1.758766830582798e-8-t969.*2.524706033578261e-9;
et65 = t4.*t7.*1.624043742404524e-7;
K = ft_3({dq1,dq2,dq3,dq4,dq5,dq6,et22,et23,et51,et52,et53,et54,et55,et56,et57,et58,et59,et60,et61,et62,et63,et64,et65,t1001,t1003,t1009,t1012,t1018,t1021,t1022,t1030,t1031,t1032,t1034,t1038,t1039,t1041,t1050,t1054,t1059,t1072,t1078,t1083,t1090,t1091,t1103,t1106,t1107,t1108,t1109,t1111,t1113,t1114,t1115,t1116,t1117,t1119,t1121,t1122,t1124,t1125,t1127,t1128,t1129,t1130,t1131,t1132,t1135,t1137,t1138,t1139,t1140,t1141,t1142,t1143,t1144,t1145,t1146,t1151,t1153,t1156,t1157,t1158,t1164,t1167,t1168,t1170,t1171,t1173,t1174,t1175,t1176,t1177,t1178,t1179,t1180,t1182,t1183,t1189,t119,t1191,t1193,t1194,t1195,t1196,t1197,t1198,t1199,t1200,t1202,t1204,t1205,t1206,t121,t1217,t1220,t1229,t1233,t1238,t1245,t1246,t1249,t1270,t1271,t1272,t1273,t1274,t1280,t1284,t1285,t1287,t1289,t1294,t1296,t1305,t1308,t1315,t1319,t1323,t1325,t1329,t1331,t1340,t1341,t1342,t1343,t1346,t1347,t1348,t135,t1360,t1365,t1384,t1392,t1394,t14,t1403,t1405,t1409,t141,t1412,t1413,t1414,t1417,t1418,t1419,t1420,t1421,t1422,t1424,t1425,t1426,t1430,t1432,t1433,t1434,t1435,t1436,t15,t150,t154,t16,t161,t163,t168,t169,t17,t171,t172,t177,t18,t180,t181,t184,t186,t19,t191,t196,t2,t20,t200,t21,t217,t218,t219,t227,t232,t233,t234,t241,t246,t248,t251,t255,t257,t258,t26,t260,t261,t262,t267,t268,t27,t273,t278,t282,t287,t288,t289,t291,t292,t294,t295,t296,t298,t3,t30,t302,t303,t305,t307,t315,t316,t319,t321,t322,t326,t327,t328,t329,t331,t332,t334,t336,t337,t341,t343,t344,t345,t346,t347,t348,t349,t35,t351,t353,t354,t355,t356,t357,t362,t364,t365,t366,t368,t374,t379,t38,t380,t386,t388,t392,t396,t397,t399,t4,t404,t405,t406,t407,t410,t417,t425,t427,t429,t443,t444,t449,t450,t451,t453,t457,t460,t467,t47,t473,t476,t481,t488,t498,t5,t503,t505,t507,t513,t520,t523,t524,t526,t531,t546,t555,t568,t570,t571,t572,t579,t581,t584,t585,t586,t587,t588,t589,t590,t592,t593,t596,t599,t6,t600,t602,t604,t605,t606,t607,t608,t609,t610,t614,t615,t617,t618,t619,t62,t620,t622,t623,t624,t625,t626,t627,t628,t629,t631,t635,t637,t638,t639,t640,t641,t642,t643,t644,t649,t650,t652,t653,t654,t656,t659,t660,t664,t665,t666,t669,t670,t672,t673,t674,t675,t682,t697,t7,t701,t704,t71,t713,t714,t719,t72,t722,t732,t738,t74,t75,t757,t758,t763,t768,t769,t772,t775,t777,t781,t782,t788,t795,t798,t8,t803,t813,t816,t818,t822,t823,t825,t831,t835,t839,t843,t845,t847,t854,t856,t858,t860,t862,t864,t869,t870,t871,t879,t888,t892,t893,t9,t90,t903,t907,t913,t918,t923,t925,t928,t932,t933,t938,t947,t948,t964,t965,t966,t968,t969,t970,t972,t973,t976,t980,t985,t986,t995});
end
function K = ft_3(ct)
dq1 = ct{1};
dq2 = ct{2};
dq3 = ct{3};
dq4 = ct{4};
dq5 = ct{5};
dq6 = ct{6};
et22 = ct{7};
et23 = ct{8};
et51 = ct{9};
et52 = ct{10};
et53 = ct{11};
et54 = ct{12};
et55 = ct{13};
et56 = ct{14};
et57 = ct{15};
et58 = ct{16};
et59 = ct{17};
et60 = ct{18};
et61 = ct{19};
et62 = ct{20};
et63 = ct{21};
et64 = ct{22};
et65 = ct{23};
t1001 = ct{24};
t1003 = ct{25};
t1009 = ct{26};
t1012 = ct{27};
t1018 = ct{28};
t1021 = ct{29};
t1022 = ct{30};
t1030 = ct{31};
t1031 = ct{32};
t1032 = ct{33};
t1034 = ct{34};
t1038 = ct{35};
t1039 = ct{36};
t1041 = ct{37};
t1050 = ct{38};
t1054 = ct{39};
t1059 = ct{40};
t1072 = ct{41};
t1078 = ct{42};
t1083 = ct{43};
t1090 = ct{44};
t1091 = ct{45};
t1103 = ct{46};
t1106 = ct{47};
t1107 = ct{48};
t1108 = ct{49};
t1109 = ct{50};
t1111 = ct{51};
t1113 = ct{52};
t1114 = ct{53};
t1115 = ct{54};
t1116 = ct{55};
t1117 = ct{56};
t1119 = ct{57};
t1121 = ct{58};
t1122 = ct{59};
t1124 = ct{60};
t1125 = ct{61};
t1127 = ct{62};
t1128 = ct{63};
t1129 = ct{64};
t1130 = ct{65};
t1131 = ct{66};
t1132 = ct{67};
t1135 = ct{68};
t1137 = ct{69};
t1138 = ct{70};
t1139 = ct{71};
t1140 = ct{72};
t1141 = ct{73};
t1142 = ct{74};
t1143 = ct{75};
t1144 = ct{76};
t1145 = ct{77};
t1146 = ct{78};
t1151 = ct{79};
t1153 = ct{80};
t1156 = ct{81};
t1157 = ct{82};
t1158 = ct{83};
t1164 = ct{84};
t1167 = ct{85};
t1168 = ct{86};
t1170 = ct{87};
t1171 = ct{88};
t1173 = ct{89};
t1174 = ct{90};
t1175 = ct{91};
t1176 = ct{92};
t1177 = ct{93};
t1178 = ct{94};
t1179 = ct{95};
t1180 = ct{96};
t1182 = ct{97};
t1183 = ct{98};
t1189 = ct{99};
t119 = ct{100};
t1191 = ct{101};
t1193 = ct{102};
t1194 = ct{103};
t1195 = ct{104};
t1196 = ct{105};
t1197 = ct{106};
t1198 = ct{107};
t1199 = ct{108};
t1200 = ct{109};
t1202 = ct{110};
t1204 = ct{111};
t1205 = ct{112};
t1206 = ct{113};
t121 = ct{114};
t1217 = ct{115};
t1220 = ct{116};
t1229 = ct{117};
t1233 = ct{118};
t1238 = ct{119};
t1245 = ct{120};
t1246 = ct{121};
t1249 = ct{122};
t1270 = ct{123};
t1271 = ct{124};
t1272 = ct{125};
t1273 = ct{126};
t1274 = ct{127};
t1280 = ct{128};
t1284 = ct{129};
t1285 = ct{130};
t1287 = ct{131};
t1289 = ct{132};
t1294 = ct{133};
t1296 = ct{134};
t1305 = ct{135};
t1308 = ct{136};
t1315 = ct{137};
t1319 = ct{138};
t1323 = ct{139};
t1325 = ct{140};
t1329 = ct{141};
t1331 = ct{142};
t1340 = ct{143};
t1341 = ct{144};
t1342 = ct{145};
t1343 = ct{146};
t1346 = ct{147};
t1347 = ct{148};
t1348 = ct{149};
t135 = ct{150};
t1360 = ct{151};
t1365 = ct{152};
t1384 = ct{153};
t1392 = ct{154};
t1394 = ct{155};
t14 = ct{156};
t1403 = ct{157};
t1405 = ct{158};
t1409 = ct{159};
t141 = ct{160};
t1412 = ct{161};
t1413 = ct{162};
t1414 = ct{163};
t1417 = ct{164};
t1418 = ct{165};
t1419 = ct{166};
t1420 = ct{167};
t1421 = ct{168};
t1422 = ct{169};
t1424 = ct{170};
t1425 = ct{171};
t1426 = ct{172};
t1430 = ct{173};
t1432 = ct{174};
t1433 = ct{175};
t1434 = ct{176};
t1435 = ct{177};
t1436 = ct{178};
t15 = ct{179};
t150 = ct{180};
t154 = ct{181};
t16 = ct{182};
t161 = ct{183};
t163 = ct{184};
t168 = ct{185};
t169 = ct{186};
t17 = ct{187};
t171 = ct{188};
t172 = ct{189};
t177 = ct{190};
t18 = ct{191};
t180 = ct{192};
t181 = ct{193};
t184 = ct{194};
t186 = ct{195};
t19 = ct{196};
t191 = ct{197};
t196 = ct{198};
t2 = ct{199};
t20 = ct{200};
t200 = ct{201};
t21 = ct{202};
t217 = ct{203};
t218 = ct{204};
t219 = ct{205};
t227 = ct{206};
t232 = ct{207};
t233 = ct{208};
t234 = ct{209};
t241 = ct{210};
t246 = ct{211};
t248 = ct{212};
t251 = ct{213};
t255 = ct{214};
t257 = ct{215};
t258 = ct{216};
t26 = ct{217};
t260 = ct{218};
t261 = ct{219};
t262 = ct{220};
t267 = ct{221};
t268 = ct{222};
t27 = ct{223};
t273 = ct{224};
t278 = ct{225};
t282 = ct{226};
t287 = ct{227};
t288 = ct{228};
t289 = ct{229};
t291 = ct{230};
t292 = ct{231};
t294 = ct{232};
t295 = ct{233};
t296 = ct{234};
t298 = ct{235};
t3 = ct{236};
t30 = ct{237};
t302 = ct{238};
t303 = ct{239};
t305 = ct{240};
t307 = ct{241};
t315 = ct{242};
t316 = ct{243};
t319 = ct{244};
t321 = ct{245};
t322 = ct{246};
t326 = ct{247};
t327 = ct{248};
t328 = ct{249};
t329 = ct{250};
t331 = ct{251};
t332 = ct{252};
t334 = ct{253};
t336 = ct{254};
t337 = ct{255};
t341 = ct{256};
t343 = ct{257};
t344 = ct{258};
t345 = ct{259};
t346 = ct{260};
t347 = ct{261};
t348 = ct{262};
t349 = ct{263};
t35 = ct{264};
t351 = ct{265};
t353 = ct{266};
t354 = ct{267};
t355 = ct{268};
t356 = ct{269};
t357 = ct{270};
t362 = ct{271};
t364 = ct{272};
t365 = ct{273};
t366 = ct{274};
t368 = ct{275};
t374 = ct{276};
t379 = ct{277};
t38 = ct{278};
t380 = ct{279};
t386 = ct{280};
t388 = ct{281};
t392 = ct{282};
t396 = ct{283};
t397 = ct{284};
t399 = ct{285};
t4 = ct{286};
t404 = ct{287};
t405 = ct{288};
t406 = ct{289};
t407 = ct{290};
t410 = ct{291};
t417 = ct{292};
t425 = ct{293};
t427 = ct{294};
t429 = ct{295};
t443 = ct{296};
t444 = ct{297};
t449 = ct{298};
t450 = ct{299};
t451 = ct{300};
t453 = ct{301};
t457 = ct{302};
t460 = ct{303};
t467 = ct{304};
t47 = ct{305};
t473 = ct{306};
t476 = ct{307};
t481 = ct{308};
t488 = ct{309};
t498 = ct{310};
t5 = ct{311};
t503 = ct{312};
t505 = ct{313};
t507 = ct{314};
t513 = ct{315};
t520 = ct{316};
t523 = ct{317};
t524 = ct{318};
t526 = ct{319};
t531 = ct{320};
t546 = ct{321};
t555 = ct{322};
t568 = ct{323};
t570 = ct{324};
t571 = ct{325};
t572 = ct{326};
t579 = ct{327};
t581 = ct{328};
t584 = ct{329};
t585 = ct{330};
t586 = ct{331};
t587 = ct{332};
t588 = ct{333};
t589 = ct{334};
t590 = ct{335};
t592 = ct{336};
t593 = ct{337};
t596 = ct{338};
t599 = ct{339};
t6 = ct{340};
t600 = ct{341};
t602 = ct{342};
t604 = ct{343};
t605 = ct{344};
t606 = ct{345};
t607 = ct{346};
t608 = ct{347};
t609 = ct{348};
t610 = ct{349};
t614 = ct{350};
t615 = ct{351};
t617 = ct{352};
t618 = ct{353};
t619 = ct{354};
t62 = ct{355};
t620 = ct{356};
t622 = ct{357};
t623 = ct{358};
t624 = ct{359};
t625 = ct{360};
t626 = ct{361};
t627 = ct{362};
t628 = ct{363};
t629 = ct{364};
t631 = ct{365};
t635 = ct{366};
t637 = ct{367};
t638 = ct{368};
t639 = ct{369};
t640 = ct{370};
t641 = ct{371};
t642 = ct{372};
t643 = ct{373};
t644 = ct{374};
t649 = ct{375};
t650 = ct{376};
t652 = ct{377};
t653 = ct{378};
t654 = ct{379};
t656 = ct{380};
t659 = ct{381};
t660 = ct{382};
t664 = ct{383};
t665 = ct{384};
t666 = ct{385};
t669 = ct{386};
t670 = ct{387};
t672 = ct{388};
t673 = ct{389};
t674 = ct{390};
t675 = ct{391};
t682 = ct{392};
t697 = ct{393};
t7 = ct{394};
t701 = ct{395};
t704 = ct{396};
t71 = ct{397};
t713 = ct{398};
t714 = ct{399};
t719 = ct{400};
t72 = ct{401};
t722 = ct{402};
t732 = ct{403};
t738 = ct{404};
t74 = ct{405};
t75 = ct{406};
t757 = ct{407};
t758 = ct{408};
t763 = ct{409};
t768 = ct{410};
t769 = ct{411};
t772 = ct{412};
t775 = ct{413};
t777 = ct{414};
t781 = ct{415};
t782 = ct{416};
t788 = ct{417};
t795 = ct{418};
t798 = ct{419};
t8 = ct{420};
t803 = ct{421};
t813 = ct{422};
t816 = ct{423};
t818 = ct{424};
t822 = ct{425};
t823 = ct{426};
t825 = ct{427};
t831 = ct{428};
t835 = ct{429};
t839 = ct{430};
t843 = ct{431};
t845 = ct{432};
t847 = ct{433};
t854 = ct{434};
t856 = ct{435};
t858 = ct{436};
t860 = ct{437};
t862 = ct{438};
t864 = ct{439};
t869 = ct{440};
t870 = ct{441};
t871 = ct{442};
t879 = ct{443};
t888 = ct{444};
t892 = ct{445};
t893 = ct{446};
t9 = ct{447};
t90 = ct{448};
t903 = ct{449};
t907 = ct{450};
t913 = ct{451};
t918 = ct{452};
t923 = ct{453};
t925 = ct{454};
t928 = ct{455};
t932 = ct{456};
t933 = ct{457};
t938 = ct{458};
t947 = ct{459};
t948 = ct{460};
t964 = ct{461};
t965 = ct{462};
t966 = ct{463};
t968 = ct{464};
t969 = ct{465};
t970 = ct{466};
t972 = ct{467};
t973 = ct{468};
t976 = ct{469};
t980 = ct{470};
t985 = ct{471};
t986 = ct{472};
t995 = ct{473};
et66 = t7.*t8.*3.561624112004214e-7;
et67 = t4.*t71.*6.903101118415674e-6;
et68 = t4.*t75.*5.419930569269819e-6;
et69 = t8.*t71.*(-3.147703918772038e-6);
et70 = t8.*t75.*1.18862287368685e-5;
et71 = t3.*t30.*t72.*1.509062034684317e-22+t4.*t30.*t72.*2.409335246872506e-25;
et72 = t3.*t4.*t30.*t72.*6.078930528964336e-22;
et73 = t3.*t8.*t30.*t72.*1.333145467812469e-21;
et74 = t8.*6.806468937857363e-8+t75.*2.616246e-7;
et75 = t964.*8.01825475553694e-7+t965.*4.35810366141993e-7;
et76 = t4.*t7.*1.144847168350722e-7;
et77 = t4.*t75.*3.820705072696559e-6;
et78 = t8.*t71.*(-2.218930330581593e-6)+t5.*t1413+t9.*t1414+t5.*(t531-t969).*4.35810366141993e-7;
et79 = t9.*(t531-t969).*(-8.01825475553694e-7)+t1341.*(et62+et63+et64+et65+et66+et67+et68+et69+et70+et71+et72+et73)+t3.*t30.*t72.*1.484360353741602e-23;
et80 = t3.*t4.*t30.*t72.*4.285257977338449e-22;
et81 = (dq1.*t1434)./2.0+(dq6.*(et53+et54))./2.0+(dq5.*(t5.*8.01825475553694e-7+t9.*4.35810366141993e-7+t5.*t364+t9.*t368+t1340.*(et55+et56)+2.616246e-7))./2.0;
et82 = (dq4.*(t4.*t5.*4.35810366141993e-7-t4.*t9.*8.01825475553694e-7-t5.*t714+t9.*t738+t181.*t1341))./2.0-(dq3.*(et57+et58+et59+et60+et61))./2.0+(dq2.*(et74+et75+et76+et77+et78+et79+et80))./2.0;
et83 = t74.*(-3.87668616986977e-7)+t388+t392+t405+t427-t585-t590-t593-t605+t606+t617+t1018+t1022+t1054+t1128+t1138+t1174;
et84 = t2.*t75.*(-4.395308215012666e-6);
et85 = t4.*t74.*1.200790562256725e-5+t4.*t75.*6.359001115808088e-7;
et86 = t5.*t74.*2.10868590222219e-13-t8.*t71.*1.069583140309415e-6;
et87 = t5.*t75.*(-6.429626140715183e-6);
et88 = t6.*t75.*(-1.813078608102233e-5)-t7.*t74.*3.40807331083027e-6;
et89 = t8.*t74.*(-9.33523109899656e-6)+t9.*t74.*1.608000198040319e-13;
et90 = t9.*t75.*1.182954431201322e-5+t17.*t74.*7.452372645815517e-7;
et91 = t30.*t72.*1.74829743798322e-20;
et92 = t2.*t4.*t74.*3.5155453823114e-6+t4.*t5.*t71.*2.7046541903611e-13;
et93 = t2.*t5.*t75.*(-1.882396747564322e-6);
et94 = t2.*t8.*t74.*(-2.733068497907686e-6)-t4.*t5.*t75.*2.227142959217101e-7;
et95 = t4.*t6.*t74.*1.4501736435025e-5;
et96 = t4.*t9.*t71.*(-3.546806877605634e-13)+t5.*t8.*t71.*3.746051489620971e-7;
et97 = t2.*t9.*t75.*3.46332667728404e-6+t4.*t8.*t74.*3.016314764575132e-7;
et98 = t5.*t6.*t75.*(-7.764946411068142e-6)+t5.*t7.*t74.*1.378434177095879e-6;
et99 = t5.*t8.*t74.*(-1.182954431201322e-5)+t4.*t9.*t75.*4.097607815548108e-7;
et100 = t6.*t8.*t74.*(-1.12739944177504e-5)-t8.*t9.*t71.*6.892170885479394e-7;
et101 = t6.*t9.*t75.*1.428633261714363e-5+t7.*t9.*t74.*7.492102979241942e-7;
et102 = t8.*t9.*t74.*(-6.429626140715183e-6)-t8.*t9.*t75.*2.10868590222219e-13;
et103 = t8.*t16.*t71.*2.139166280618831e-6-t5.*t17.*t74.*4.217371804444381e-13;
et104 = t4.*t18.*t75.*(-1.274380648825446e-6)+t8.*t18.*t71.*2.143506553146841e-6;
et105 = t7.*t17.*t74.*5.073437414621283e-7+t7.*t18.*t74.*2.817872251232979e-6;
et106 = t9.*t17.*t74.*(-3.216000396080637e-13);
et107 = t2.*t30.*t72.*5.325743171835082e-21;
et108 = t4.*t30.*t72.*1.185912239144439e-21;
et109 = t5.*t30.*t72.*(-7.82072115054759e-23);
et110 = t6.*t30.*t72.*2.196885984950864e-20;
et111 = t7.*t30.*t72.*(-3.845355261323178e-23);
et112 = t8.*t30.*t72.*1.525438641344884e-21;
et113 = t9.*t30.*t72.*(-4.25073965847863e-23);
et114 = t16.*t30.*t72.*(-1.933613622435097e-22);
et115 = t17.*t30.*t72.*(-5.756958141897304e-23);
et116 = t18.*t30.*t72.*(-7.993777824483687e-23)+t5.*t75.*t135;
et117 = t2.*t5.*t8.*t74.*(-3.46332667728404e-6)-t4.*t5.*t8.*t74.*8.195215631096216e-7;
et118 = t2.*t8.*t9.*t74.*(-1.882396747564322e-6)+t4.*t5.*t9.*t75.*8.376559107229145e-7;
et119 = t4.*t7.*t8.*t74.*(-1.253488085959302e-6)-t5.*t6.*t8.*t74.*1.428633261714363e-5;
et120 = t5.*t8.*t9.*t71.*(-1.408936125616489e-6)-t4.*t8.*t9.*t74.*4.454285918434201e-7;
et121 = t5.*t7.*t9.*t74.*4.287013106293682e-6-t4.*t5.*t16.*t71.*5.4093083807222e-13;
et122 = t6.*t8.*t9.*t74.*(-7.764946411068142e-6)+t4.*t9.*t16.*t71.*7.093613755211269e-13;
et123 = t5.*t8.*t16.*t71.*(-7.492102979241942e-7)-t5.*t7.*t17.*t74.*1.378434177095879e-6;
et124 = t4.*t8.*t18.*t74.*(-8.376559107229145e-7)+t8.*t9.*t16.*t71.*1.378434177095879e-6;
et125 = t2.*t3.*t30.*t72.*(-2.49373386785477e-22);
et126 = t7.*t9.*t17.*t74.*(-7.492102979241942e-7);
et127 = t2.*t4.*t30.*t72.*2.608176229845321e-22;
et128 = t3.*t4.*t30.*t72.*(-6.599207038311596e-23);
et129 = t3.*t5.*t30.*t72.*(-2.298746926034785e-23);
et130 = t3.*t6.*t30.*t72.*(-1.028673146211772e-21);
et131 = t4.*t5.*t30.*t72.*1.502780299100031e-21;
et132 = t2.*t8.*t30.*t72.*3.354896486533935e-22;
et133 = t4.*t6.*t30.*t72.*1.075880984259862e-21;
et134 = t4.*t7.*t30.*t72.*(-4.293116821085015e-23);
et135 = t8.*t16.*t18.*t71.*(-4.287013106293682e-6);
et136 = t3.*t9.*t30.*t72.*4.229348336668283e-23;
et137 = t4.*t8.*t30.*t72.*1.42236473075195e-22;
et138 = t5.*t7.*t30.*t72.*2.188339739859402e-29;
et139 = t4.*t9.*t30.*t72.*8.167952407966379e-22;
et140 = t5.*t9.*t30.*t72.*(-1.216145632129581e-22);
et141 = t6.*t8.*t30.*t72.*1.383905463411169e-21;
et142 = t7.*t17.*t18.*t74.*(-1.408936125616489e-6);
et143 = t7.*t8.*t30.*t72.*3.337571006928825e-23;
et144 = t7.*t9.*t30.*t72.*1.66874105402097e-29;
et145 = t5.*t16.*t30.*t72.*7.82072115054759e-23;
et146 = t5.*t17.*t30.*t72.*1.564144230109518e-22;
et147 = t7.*t17.*t30.*t72.*7.733879758902498e-23;
et148 = t9.*t16.*t30.*t72.*4.25073965847863e-23;
et149 = t9.*t17.*t30.*t72.*8.501479316957259e-23;
et150 = t16.*t17.*t30.*t72.*2.878479070948652e-23;
et151 = t16.*t18.*t30.*t72.*1.598755564896737e-22;
et152 = t17.*t18.*t30.*t72.*1.598755564896737e-22;
et153 = t4.*t5.*t7.*t8.*t74.*7.093613755211269e-13-t4.*t5.*t8.*t9.*t74.*1.274380648825446e-6;
et154 = t4.*t7.*t8.*t9.*t74.*5.4093083807222e-13+t5.*t8.*t9.*t16.*t71.*2.817872251232979e-6;
et155 = t2.*t3.*t5.*t30.*t72.*(-1.068001671898062e-22);
et156 = t5.*t7.*t9.*t17.*t74.*(-2.143506553146841e-6);
et157 = t2.*t4.*t5.*t30.*t72.*3.305064005090484e-22;
et158 = t3.*t4.*t5.*t30.*t72.*2.311271412620895e-23;
et159 = t2.*t4.*t7.*t30.*t72.*(-1.994589265414034e-22);
et160 = t2.*t3.*t9.*t30.*t72.*1.964962320751208e-22;
et161 = t3.*t5.*t6.*t30.*t72.*(-4.405540840394095e-22);
et162 = t2.*t4.*t9.*t30.*t72.*1.79637738896555e-22;
et163 = t4.*t5.*t6.*t30.*t72.*1.363349406435421e-21;
et164 = t3.*t4.*t9.*t30.*t72.*(-4.252391506801831e-23);
et165 = t3.*t5.*t8.*t30.*t72.*(-1.66874105402097e-29);
et166 = t2.*t7.*t8.*t30.*t72.*1.550641079758662e-22;
et167 = t4.*t5.*t8.*t30.*t72.*(-8.04930348521637e-29);
et168 = t4.*t6.*t7.*t30.*t72.*(-8.227744112962308e-22);
et169 = t3.*t6.*t9.*t30.*t72.*8.105532024608353e-22;
et170 = t3.*t7.*t8.*t30.*t72.*(-1.213683123456844e-22);
et171 = t4.*t6.*t9.*t30.*t72.*7.4101138229338e-22;
et172 = t4.*t7.*t8.*t30.*t72.*3.130253519639126e-23;
et173 = t3.*t8.*t9.*t30.*t72.*2.188339739859402e-29;
et174 = t5.*t7.*t8.*t30.*t72.*4.229348336668283e-23;
et175 = t4.*t8.*t9.*t30.*t72.*(-6.138079447808974e-29);
et176 = t6.*t7.*t8.*t30.*t72.*6.396443737329302e-22;
et177 = t7.*t8.*t9.*t30.*t72.*2.298746926034785e-23;
et178 = t3.*t4.*t18.*t30.*t72.*1.32251930673679e-22;
et179 = t4.*t8.*t16.*t30.*t72.*(-7.111823653759751e-23);
et180 = t5.*t7.*t17.*t30.*t72.*(-4.376679479718804e-29);
et181 = t5.*t9.*t16.*t30.*t72.*2.432291264259161e-22;
et182 = t5.*t9.*t17.*t30.*t72.*2.432291264259161e-22;
et183 = t7.*t9.*t17.*t30.*t72.*(-3.337482108041939e-29);
et184 = t5.*t16.*t17.*t30.*t72.*(-7.82072115054759e-23);
et185 = t9.*t16.*t17.*t30.*t72.*(-4.25073965847863e-23);
et186 = t16.*t17.*t18.*t30.*t72.*(-7.993777824483687e-23);
et187 = t3.*t4.*t5.*t7.*t30.*t72.*3.069039723904487e-29;
et188 = t3.*t4.*t5.*t9.*t30.*t72.*(-8.69297658713101e-23);
et189 = t2.*t5.*t7.*t8.*t30.*t72.*1.964962320751208e-22;
et190 = t3.*t4.*t7.*t9.*t30.*t72.*(-4.024651742608185e-29);
et191 = t3.*t5.*t7.*t8.*t30.*t72.*4.25073965847863e-23;
et192 = t4.*t5.*t7.*t8.*t30.*t72.*(-8.504783013603662e-23);
et193 = t2.*t7.*t8.*t9.*t30.*t72.*1.068001671898062e-22;
et194 = t5.*t6.*t7.*t8.*t30.*t72.*8.105532024608353e-22;
et195 = t3.*t7.*t8.*t9.*t30.*t72.*(-7.82072115054759e-23);
et196 = t4.*t7.*t8.*t9.*t30.*t72.*(-4.62254282524179e-23);
et197 = t6.*t7.*t8.*t9.*t30.*t72.*4.405540840394095e-22;
et198 = t4.*t5.*t8.*t16.*t30.*t72.*4.024651742608185e-29;
et199 = t3.*t7.*t8.*t18.*t30.*t72.*2.432291264259161e-22;
et200 = t4.*t7.*t8.*t18.*t30.*t72.*(-8.69297658713101e-23);
et201 = t4.*t8.*t9.*t16.*t30.*t72.*3.069039723904487e-29;
et202 = t5.*t9.*t16.*t17.*t30.*t72.*(-1.216145632129581e-22);
et203 = t3.*t5.*t7.*t8.*t9.*t30.*t72.*(-1.598755564896737e-22);
et204 = t4.*t5.*t7.*t8.*t9.*t30.*t72.*(-1.32251930673679e-22);
et205 = t9.*(t1325+(t47.*t1249.*(t1289+t5.*(t649-t1220)))./1.316403645856965e+67+(t1249.*t1347.*(t26-t27))./1.316403645856965e+67);
et206 = -1.40259855e-11;
et207 = t1270+t5.*(-t1360+t1246.*(t965+t5.*(t531-t969))+(t1249.*t1346.*(t26-t27))./1.316403645856965e+67).*1.40259855e-11+et205.*et206+t121.*t186+t357.*t364+t356.*t368;
et208 = t355.*(t1274-t1348+(t1249.*t1294.*(t26-t27))./1.316403645856965e+67);
et209 = t5.*4.097607815548108e-7+t7.*6.685859772666872e-9;
et210 = t9.*2.227142959217101e-7-t14.*5.859823945197205e-8;
et211 = t15.*(-2.094139776807286e-7)-t21.*3.185951622063616e-7+t141+t154+t163+t171+t180+t184+t233+t255+t262+t273+t288+t302+t362;
et212 = t3.*t4.*(-2.170136264005124e-9)-t5.*t14.*4.097607815548108e-7;
et213 = t7.*t14.*(-6.267440429796511e-7)-t9.*t14.*2.227142959217101e-7;
et214 = t5.*t20.*2.10868590222219e-13+t7.*t20.*9.856216067305823e-8;
et215 = t9.*t20.*1.608000198040319e-13-t14.*t15.*2.094139776807286e-7;
et216 = t14.*t21.*(-3.185951622063616e-7)-t3.*t4.*t15.*1.07175327657342e-6;
et217 = t5.*t7.*t14.*3.546806877605634e-13+t3.*t4.*t21.*7.044680628082447e-7;
et218 = t7.*t9.*t14.*2.7046541903611e-13+t5.*t7.*t20.*6.892170885479394e-7;
et219 = t7.*t9.*t20.*3.746051489620971e-7+t7.*t15.*t20.*3.522340314041224e-7;
et220 = t7.*t20.*t21.*5.358766382867102e-7+4.616668164022386e-6;
et221 = t3.*(-2.844856587289647e-6);
et222 = t4.*8.940013971103833e-6;
et223 = t5.*4.188040994443703e-7;
et224 = t7.*6.474095421643823e-7;
et225 = t8.*1.149953792156111e-5;
et226 = t9.*2.276295446893622e-7;
et227 = t16.*(-2.929443421869778e-6);
et228 = t17.*(-2.81948171692439e-7);
et229 = t18.*(-1.211065105878372e-6);
et230 = t19.*1.250511956078399e-9;
et231 = t20.*3.483029800032151e-7;
et232 = t21.*(-9.212362233958261e-7);
et233 = t3.*t4.*1.093188572509221e-6;
et234 = t3.*t5.*(-3.660776353481749e-6);
et235 = t4.*t5.*1.132872773043163e-5;
et236 = t3.*t8.*(-1.545129867076994e-8);
et237 = t4.*t7.*(-6.836829388815001e-6);
et238 = t3.*t9.*6.735277470591094e-6;
et239 = t5.*t7.*(-3.625084017661248e-13);
et240 = t4.*t9.*6.157420948384101e-6;
et241 = t7.*t8.*5.315113587256377e-6;
et242 = t7.*t9.*(-2.764345231392299e-13);
et243 = t5.*t16.*1.184846851663018e-6;
et244 = t5.*t17.*7.660427522186475e-7;
et245 = t7.*t17.*(-1.281152254279884e-6);
et246 = t9.*t16.*6.439911875946239e-7;
et247 = t9.*t17.*4.163616429052617e-7;
et248 = t16.*t17.*4.360923755161119e-7;
et249 = t16.*t18.*2.422130211756745e-6;
et250 = t17.*t18.*7.829937223708732e-7;
et251 = t3.*t4.*t5.*(-3.828725908394669e-7);
et252 = t3.*t4.*t7.*(-2.598906377458728e-8);
et253 = t3.*t4.*t9.*7.044279371874937e-7;
et254 = t3.*t5.*t8.*2.764345231392299e-13;
et255 = t4.*t5.*t8.*(-3.94216241479634e-13);
et256 = t3.*t7.*t8.*(-1.838741722230682e-6);
et257 = t4.*t7.*t8.*(-5.185406908527248e-7);
et258 = t3.*t8.*t9.*(-3.625084017661248e-13);
et259 = t5.*t7.*t8.*6.735277470591094e-6;
et260 = t4.*t8.*t9.*(-3.006136635626675e-13);
et261 = t7.*t8.*t9.*3.660776353481749e-6;
et262 = t3.*t4.*t18.*(-2.190813206274814e-6);
et263 = t4.*t8.*t16.*(-1.077448192248847e-6);
et264 = t5.*t7.*t17.*7.250168035322496e-13;
et265 = t5.*t9.*t16.*3.684944893583304e-6;
et266 = t5.*t9.*t17.*1.191219491402018e-6;
et267 = t7.*t9.*t17.*5.528690462784599e-13;
et268 = t5.*t16.*t17.*(-1.184846851663018e-6);
et269 = t9.*t16.*t17.*(-6.439911875946239e-7);
et270 = t16.*t17.*t18.*(-1.211065105878372e-6);
et271 = t3.*t4.*t5.*t7.*4.649624995570082e-13;
et272 = t3.*t4.*t5.*t9.*1.440030993265091e-6;
et273 = t3.*t4.*t7.*t9.*(-6.097386487095885e-13);
et274 = t3.*t5.*t7.*t8.*6.439911875946239e-7;
et275 = t4.*t5.*t7.*t8.*1.408855874374987e-6;
et276 = t3.*t7.*t8.*t9.*(-1.184846851663018e-6);
et277 = t4.*t7.*t8.*t9.*7.657451816789338e-7;
et278 = t4.*t5.*t8.*t16.*6.097386487095885e-13;
et279 = t3.*t7.*t8.*t18.*3.684944893583304e-6;
et280 = t4.*t7.*t8.*t18.*1.440030993265091e-6;
et281 = t4.*t8.*t9.*t16.*4.649624995570082e-13;
et282 = t5.*t9.*t16.*t17.*(-1.842472446791652e-6);
et283 = t3.*t5.*t7.*t8.*t9.*(-2.422130211756745e-6);
et284 = t4.*t5.*t7.*t8.*t9.*2.190813206274814e-6;
et285 = 8.99453681175877e-5;
et286 = t1422.*(t1325+(t47.*t1249.*(t1289+t5.*(t649-t1220)))./1.316403645856965e+67+(t1249.*t1347.*(t26-t27))./1.316403645856965e+67)+t121.*t1433-t356.*t1432;
et287 = -t1430.*(t1274-t1348+(t1249.*t1294.*(t26-t27))./1.316403645856965e+67)-t357.*(-t1238+t1296+t1305+t1323+t1329+t1392+t1394+t1403+t1405);
et288 = (-t1360+t1246.*(t965+t5.*(t531-t969))+(t1249.*t1346.*(t26-t27))./1.316403645856965e+67).*(t1229-t1308+t1315+t1319-t1409+t1287.*(t1289+t5.*(t649-t1220)).*1.40259855e-11);
et289 = t964.*(-1.40259855e-11)+t968.*7.26350610236655e-5;
et290 = t4.*t5.*(-1.134411489642894e-5);
et291 = t3.*t9.*1.908078613917869e-5;
et292 = t9.*t74.*6.367841787827598e-4+t9.*(t531-t969).*1.40259855e-11;
et293 = t5.*t7.*t8.*1.908078613917869e-5;
et294 = t4.*t5.*t71.*3.698217217635989e-4+t4.*t9.*t74.*4.36041e-5;
et295 = t5.*t8.*t75.*6.367841787827598e-4;
et296 = t8.*t30.*t72.*6.93158769201428e-21;
et297 = t7.*t9.*t30.*t72.*(-7.142096628897415e-20);
et298 = t8.*t9.*t30.*t72.*4.161153561678485e-21;
et299 = t3.*t5.*t8.*t30.*t72.*7.142096628897415e-20;
et300 = t4.*t7.*t9.*t30.*t72.*(-2.47393392290267e-21);
et301 = t8.*1.134411489642894e-5+t75.*4.36041e-5;
et302 = t4.*t7.*1.908078613917869e-5;
et303 = t4.*t75.*6.367841787827598e-4;
et304 = t8.*t71.*(-3.698217217635989e-4)+t35.*t948+t38.*t948+t5.*(t531-t969).*7.26350610236655e-5;
et305 = t9.*(t531-t969).*(-1.33637579258949e-4)+t3.*t30.*t72.*2.47393392290267e-21;
et306 = t3.*t4.*t30.*t72.*7.142096628897415e-20;
et307 = t965.*1.40259855e-11+t968.*1.33637579258949e-4;
et308 = t3.*t5.*1.908078613917869e-5;
et309 = t4.*t9.*1.134411489642894e-5;
et310 = t5.*t74.*6.367841787827598e-4+t5.*(t531-t969).*1.40259855e-11;
et311 = t7.*t8.*t9.*(-1.908078613917869e-5)+t4.*t5.*t74.*4.36041e-5;
et312 = t4.*t9.*t71.*(-3.698217217635989e-4);
et313 = t8.*t9.*t75.*(-6.367841787827598e-4);
et314 = t8.*t30.*t72.*1.275307801118396e-20;
et315 = t5.*t7.*t30.*t72.*(-7.142096628897415e-20);
et316 = t5.*t8.*t30.*t72.*4.161153561678485e-21-t4.*t5.*t7.*t30.*t72.*2.47393392290267e-21;
et317 = t3.*t8.*t9.*t30.*t72.*(-7.142096628897415e-20);
et318 = t74.*(-3.876686599935835e-7)+t388+t392+t405+t427+t606+t617+t1018+t1022+t1054+t1174;
et319 = -(-t1360+t1246.*(t965+t5.*(t531-t969))+(t1249.*t1346.*(t26-t27))./1.316403645856965e+67).*(et289+et290+et291+et292+et293+et294+et295+et296+et297+et298+et299+et300);
et320 = t4.*t74.*1.20079068641418e-5-t4.*t75.*1.290212831914316e-9;
et321 = t8.*t71.*2.170136264005124e-9-t7.*t74.*2.22401922077146e-6;
et322 = t8.*t74.*(-5.475413853010983e-6)+t17.*t74.*7.452373505947646e-7;
et323 = t30.*t72.*1.401374717769559e-20-t121.*t1417+t356.*t1414+t357.*t1413;
et324 = (t1274-t1348+(t1249.*t1294.*(t26-t27))./1.316403645856965e+67).*(et301+et302+et303+et304+et305+et306);
et325 = -(t1325+(t47.*t1249.*(t1289+t5.*(t649-t1220)))./1.316403645856965e+67+(t1249.*t1347.*(t26-t27))./1.316403645856965e+67).*(et307+et308+et309+et310+et311+et312+et313+et314+et315+et316+et317);
et326 = t4.*t8.*t74.*8.531618370996951e-7-t8.*t16.*t71.*4.340272528010248e-9;
et327 = t7.*t17.*t74.*1.435017073119793e-6;
et328 = t4.*t30.*t72.*6.955757424542711e-22;
et329 = t7.*t30.*t72.*(-3.845355707634627e-23);
et330 = t8.*t30.*t72.*1.525438799069791e-21;
et331 = t16.*t30.*t72.*(-1.261825515365316e-22);
et332 = t17.*t30.*t72.*(-1.628350277673685e-22)-t4.*t7.*t8.*t74.*1.253488230633412e-6;
et333 = t3.*t4.*t30.*t72.*1.338949537235126e-25;
et334 = t4.*t7.*t30.*t72.*(-4.293117264977958e-23);
et335 = t4.*t8.*t30.*t72.*1.422364894917333e-22;
et336 = t7.*t8.*t30.*t72.*1.957592943650879e-23;
et337 = t7.*t17.*t30.*t72.*7.733880651525396e-23;
et338 = t16.*t17.*t30.*t72.*8.141751388368425e-23;
et339 = t3.*t7.*t8.*t30.*t72.*2.462508672736528e-25;
et340 = t4.*t7.*t8.*t30.*t72.*8.853893084262633e-23;
et341 = t4.*t8.*t16.*t30.*t72.*(-7.111824474586663e-23);
et342 = (dq1.*(et83+et84+et85+et86+et87+et88+et89+et90+et91+et92+et93+et94+et95+et96+et97+et98+et99+et100+et101+et102+et103+et104+et105+et106+et107+et108+et109+et110+et111+et112+et113+et114+et115+et116+et117+et118+et119+et120+et121+et122+et123+et124+et125+et126+et127+et128+et129+et130+et131+et132+et133+et134+et135+et136+et137+et138+et139+et140+et141+et142+et143+et144+et145+et146+et147+et148+et149+et150+et151+et152+et153+et154+et155+et156+et157+et158+et159+et160+et161+et162+et163+et164+et165+et166+et167+et168+et169+et170+et171+et172+et173+et174+et175+et176+et177+et178+et179+et180+et181+et182+et183+et184+et185+et186+et187+et188+et189+et190+et191+et192+et193+et194+et195+et196+et197+et198+et199+et200+et201+et202+et203+et204))./2.0+(dq5.*(et207+et208))./2.0-(dq4.*(et209+et210+et211+et212+et213+et214+et215+et216+et217+et218+et219+et220))./2.0;
et343 = dq3.*(et221+et222+et223+et224+et225+et226+et227+et228+et229+et230+et231+et232+et233+et234+et235+et236+et237+et238+et239+et240+et241+et242+et243+et244+et245+et246+et247+et248+et249+et250+et251+et252+et253+et254+et255+et256+et257+et258+et259+et260+et261+et262+et263+et264+et265+et266+et267+et268+et269+et270+et271+et272+et273+et274+et275+et276+et277+et278+et279+et280+et281+et282+et283+et284+et285).*(-1.0./2.0)-(dq6.*(et286+et287+et288))./2.0+(dq2.*(et318+et319+et320+et321+et322+et323+et324+et325+et326+et327+et328+et329+et330+et331+et332+et333+et334+et335+et336+et337+et338+et339+et340+et341))./2.0;
et344 = t90+t119+t150+t161-t168+t169-t172-t177+t1331-t1365+t1246.*(t965+t5.*(t531-t969)).*7.26350610236655e-5+t47.*t1249.*(t1289+t5.*(t649-t1220)).*1.015171749786156e-71;
et345 = t1249.*t1346.*(t26-t27).*5.517689141340903e-72;
et346 = t1249.*t1347.*(t26-t27).*1.015171749786156e-71;
et347 = -t191+t334-t379-t399-t513+t523+t526-t673+t722+t775+t788-t818-t823+t925+t928+t933-t964.*3.383302988283333e-6-t965.*1.246862701090643e-6-t986-t1078+t1083+t1183+t1233;
et348 = t2.*t8.*(-7.30081420113316e-6);
et349 = t6.*t8.*1.769880715106441e-6+t9.*(t531-t969).*3.383302988283333e-6;
et350 = t2.*t4.*t5.*(-7.662598700988556e-13);
et351 = t2.*t4.*t7.*(-1.22799597575967e-5);
et352 = t2.*t3.*t9.*1.288848080425708e-12;
et353 = t4.*t5.*t6.*1.857585372652597e-13;
et354 = t4.*t6.*t7.*2.976937004352228e-6;
et355 = t3.*t6.*t9.*(-3.124456121473909e-13);
et356 = t2.*t4.*t75.*(-1.769880715106441e-6);
et357 = t2.*t8.*t71.*2.976937004352228e-6;
et358 = t2.*t9.*t74.*1.857585372652597e-13;
et359 = t4.*t6.*t75.*(-7.30081420113316e-6);
et360 = t6.*t8.*t71.*1.22799597575967e-5;
et361 = t6.*t9.*t74.*7.662598700988556e-13;
et362 = t2.*t5.*t7.*t8.*1.288848080425708e-12;
et363 = t5.*t6.*t7.*t8.*(-3.124456121473909e-13);
et364 = t2.*t4.*t5.*t71.*3.124456121473909e-13;
et365 = t4.*t5.*t6.*t71.*1.288848080425708e-12;
et366 = t2.*t5.*t8.*t75.*1.857585372652597e-13;
et367 = t5.*t6.*t8.*t75.*7.662598700988556e-13;
et368 = t2.*t3.*t4.*t30.*t72.*(-3.84506501891928e-22);
et369 = t3.*t4.*t6.*t30.*t72.*(-1.586101540900623e-21);
et370 = t2.*t7.*t9.*t30.*t72.*(-4.035603346078089e-29);
et371 = t6.*t7.*t9.*t30.*t72.*(-1.664699206432988e-28);
et372 = t2.*t3.*t5.*t8.*t30.*t72.*4.035603346078089e-29;
et373 = t3.*t5.*t6.*t8.*t30.*t72.*1.664699206432988e-28;
et374 = -t1414-t2.*t8.*3.96815841743287e-6;
et375 = t6.*t8.*9.619703863182361e-7;
et376 = t2.*t3.*t5.*(-1.288848080425708e-12);
et377 = t2.*t4.*t7.*(-6.674437170347525e-6);
et378 = t3.*t5.*t6.*3.124456121473909e-13;
et379 = t2.*t4.*t9.*(-7.662598700988556e-13);
et380 = t4.*t6.*t7.*1.618032907912407e-6;
et381 = t4.*t6.*t9.*1.857585372652597e-13;
et382 = t2.*t4.*t75.*(-9.619703863182361e-7);
et383 = t2.*t5.*t74.*(-1.857585372652597e-13);
et384 = t2.*t8.*t71.*1.618032907912407e-6;
et385 = t4.*t6.*t75.*(-3.96815841743287e-6);
et386 = t5.*t6.*t74.*(-7.662598700988556e-13);
et387 = t6.*t8.*t71.*6.674437170347525e-6;
et388 = t2.*t7.*t8.*t9.*1.288848080425708e-12;
et389 = t6.*t7.*t8.*t9.*(-3.124456121473909e-13);
et390 = t2.*t4.*t9.*t71.*3.124456121473909e-13;
et391 = t4.*t6.*t9.*t71.*1.288848080425708e-12;
et392 = t2.*t8.*t9.*t75.*1.857585372652597e-13;
et393 = t6.*t8.*t9.*t75.*7.662598700988556e-13;
et394 = t2.*t3.*t4.*t30.*t72.*(-2.089880210625419e-22);
et395 = t3.*t4.*t6.*t30.*t72.*(-8.620822290548326e-22);
et396 = t2.*t5.*t7.*t30.*t72.*4.035603346078089e-29;
et397 = t5.*t6.*t7.*t30.*t72.*1.664699206432988e-28;
et398 = t2.*t3.*t8.*t9.*t30.*t72.*4.035603346078089e-29;
et399 = t3.*t6.*t8.*t9.*t30.*t72.*1.664699206432988e-28;
et400 = dq6;
et401 = (dq6.*(t1384.*t1433+t1421.*t1432+t1420.*(-t1238+t1296+t1305+t1323+t1329+t1392+t1394+t1403+t1405)))./2.0+(dq3.*(-t1420.*t1424+t1421.*t1425+t1384.*(et344+et345+et346)))./2.0-(dq1.*(-t1384.*(t397+t407+t417+t429+t449+t450+t457+t460+t473+t481+t498+t503+t769+t781+t798+t803+t831+t843+t845+t847+t854+t856+t879+t892+t985+t995+t1009+t1012+t1030+t1032+t1038+t1050+t1417)+t1421.*(et374+et375+et376+et377+et378+et379+et380+et381+et382+et383+et384+et385+et386+et387+et388+et389+et390+et391+et392+et393+et394+et395+et396+et397+et398+et399)+t1420.*(et347+et348+et349+et350+et351+et352+et353+et354+et355+et356+et357+et358+et359+et360+et361+et362+et363+et364+et365+et366+et367+et368+et369+et370+et371+et372+et373)))./2.0+(dq5.*(-t186.*t1384+t364.*t1420+t368.*t1421))./2.0+(dq4.*(-t714.*t1420+t738.*t1421+t1091.*t1384))./2.0+(dq2.*(t1384.*t1417+t1413.*t1420+t1414.*t1421))./2.0;
et402 = t227+t241+t386+t396+t397+t406+t407+t417+t425+t429+t443+t449+t450+t457+t460+t467+t473+t481+t498+t503+t670+t697+t704+t713+t732+t769+t781+t798+t803+t816+t831+t835+t843+t845+t847+t854+t856+t862+t869+t879+t888+t892+t907+t985+t995+t1003+t1009+t1012+t1030+t1031+t1032+t1038+t1039+t1050+t1059+t4.*t74.*4.20092050615074e-6-t5.*t75.*3.146556677756745e-13+t62.*t75+t8.*t719+t8.*t768;
et403 = t5.*t8.*t74.*(-4.126305279697715e-13)-t8.*t9.*t74.*3.146556677756745e-13-t3.*t5.*t30.*t72.*1.785238843466173e-29;
et404 = t4.*t5.*t30.*t72.*3.937746659416635e-29-t4.*t7.*t30.*t72.*2.383445535530781e-22;
et405 = t3.*t9.*t30.*t72.*2.341111640349547e-29+t4.*t9.*t30.*t72.*3.002769355787804e-29;
et406 = t2.*2.821008266589887e-4;
et407 = t6.*9.795760612003476e-4+t218+t232+t234+t246+t248+t251+t257+t258+t260+t261+t267+t268+t278+t282+t287+t289+t291+t292+t294+t295+t296+t298+t303+t305+t307+t315+t316+t319+t321+t322;
et408 = t326+t327+t328+t329+t331+t332+t336+t337+t341+t343+t344+t345+t346+t347+t348+t349+t351+t353+t354+t365+t366+t374+t404+t444+t451+t453+t476+t488+t505+t507+t520+t524+t546+t555+t579+t584+t586+t587+t589+t592+t596+t599+t600+t602+t604+t607+t608+t609+t610+t614+t615+t618+t619+t620+t622+t623+t624+t625+t626+t627+t628+t629+t631+t635+t637+t638+t639+t640+t641+t642+t643+t644+t650+t652+t653+t654+t656+t659+t660+t664+t665+t666+t669+t675+t682+t701+t757+t758+t763+t772+t777+t782+t795+t813+t822+t825+t839+t858+t860+t864+t870+t871+t893+t903+t913+t918+t923+t932+t938+t947+t966+t970+t972+t976+t980+t1001+t1021+t1034+t1041+t1072+t1090+t1103+t1106+t1107+t1108+t1109+t1111+t1113+t1114+t1115+t1116+t1117+t1119+t1121+t1122+t1124+t1125+t1127+t1129+t1130+t1132+t1135+t1137+t1139+t1140+t1141+t1142+t1143+t1144+t1145+t1151+t1153+t1156+t1157+t1158+t1164+t1167+t1168+t1170+t1171+t1173+t1175+t1176+t1177+t1178+t1179+t1180+t1182+t1189+t1191+t1193+t1194+t1196+t1197+t1198+t1199+t1200+t1202;
et409 = t2.*t3.*7.556062069816369e-6;
et410 = t2.*t4.*2.793386635594598e-6;
et411 = t2.*t7.*(-8.334431886523961e-9);
et412 = t3.*t6.*3.116899618889927e-5;
et413 = t2.*t8.*3.593132588990334e-6;
et414 = t4.*t6.*1.152280865277303e-5;
et415 = t6.*t7.*(-3.437979642139428e-8);
et416 = t6.*t8.*1.482178612849474e-5;
et417 = t2.*t71.*3.95755796128007e-4;
et418 = t2.*t74.*(-1.853092799186148e-5);
et419 = t2.*t75.*2.043984759722906e-8;
et420 = t6.*t71.*(-9.594005985658975e-5);
et421 = t6.*t74.*4.492311567212771e-6;
et422 = t6.*t75.*(-4.955076390854535e-9);
et423 = t2.*t3.*t5.*3.236065815824815e-6;
et424 = t2.*t4.*t5.*3.539761430212882e-6;
et425 = t2.*t4.*t7.*6.043644226648326e-6;
et426 = t2.*t3.*t9.*(-5.953874008704457e-6);
et427 = t3.*t5.*t6.*1.334887434069505e-5;
et428 = t2.*t4.*t9.*1.923940772636472e-6;
et429 = t4.*t5.*t6.*1.460162840226632e-5;
et430 = t2.*t7.*t8.*(-4.698472598739189e-6);
et431 = t4.*t6.*t7.*2.493022451733813e-5;
et432 = t3.*t6.*t9.*(-2.455991951519339e-5);
et433 = t4.*t6.*t9.*7.93631683486574e-6;
et434 = t6.*t7.*t8.*(-1.938134879923087e-5);
et435 = t2.*t4.*t71.*1.938134879923087e-5;
et436 = t2.*t4.*t75.*(-1.482178612849474e-5);
et437 = t2.*t5.*t74.*(-7.93631683486574e-6);
et438 = t2.*t8.*t71.*2.493022451733813e-5;
et439 = t4.*t6.*t71.*(-4.698472598739189e-6);
et440 = t2.*t8.*t75.*1.152280865277303e-5;
et441 = t2.*t9.*t74.*1.460162840226632e-5;
et442 = t4.*t6.*t75.*3.593132588990334e-6;
et443 = t5.*t6.*t74.*1.923940772636472e-6;
et444 = t6.*t8.*t71.*(-6.043644226648326e-6);
et445 = t6.*t8.*t75.*(-2.793386635594598e-6);
et446 = t6.*t9.*t74.*(-3.539761430212882e-6);
et447 = t2.*t30.*t72.*4.096256460969035e-28;
et448 = t6.*t30.*t72.*(-9.930242182130862e-29);
et449 = t2.*t5.*t7.*t8.*(-5.953874008704457e-6);
et450 = t2.*t7.*t8.*t9.*(-3.236065815824815e-6);
et451 = t5.*t6.*t7.*t8.*(-2.455991951519339e-5);
et452 = t6.*t7.*t8.*t9.*(-1.334887434069505e-5);
et453 = t2.*t4.*t5.*t71.*2.455991951519339e-5;
et454 = t2.*t4.*t9.*t71.*1.334887434069505e-5;
et455 = t4.*t5.*t6.*t71.*(-5.953874008704457e-6);
et456 = t2.*t5.*t8.*t75.*1.460162840226632e-5;
et457 = t4.*t6.*t9.*t71.*(-3.236065815824815e-6);
et458 = t2.*t8.*t9.*t75.*7.93631683486574e-6;
et459 = t5.*t6.*t8.*t75.*(-3.539761430212882e-6);
et460 = t6.*t8.*t9.*t75.*(-1.923940772636472e-6);
et461 = t2.*t3.*t30.*t72.*4.440555926585153e-24;
et462 = t2.*t7.*t30.*t72.*4.02584323234086e-21;
et463 = t3.*t6.*t30.*t72.*(-1.076490112239103e-24);
et464 = t6.*t7.*t30.*t72.*(-9.759544761262319e-22);
et465 = t2.*t3.*t4.*t30.*t72.*(-3.220032337442058e-21);
et466 = t2.*t3.*t8.*t30.*t72.*2.503329636416397e-21;
et467 = t3.*t4.*t6.*t30.*t72.*7.806078855113529e-22;
et468 = t2.*t5.*t7.*t30.*t72.*1.724164458109665e-21;
et469 = t3.*t6.*t8.*t30.*t72.*(-6.068631148509608e-22);
et470 = t2.*t7.*t9.*t30.*t72.*(-3.172203081801246e-21);
et471 = t5.*t6.*t7.*t30.*t72.*(-4.179760421250838e-22);
et472 = t6.*t7.*t9.*t30.*t72.*7.690130037838559e-22;
et473 = t2.*t3.*t5.*t8.*t30.*t72.*3.172203081801246e-21;
et474 = t2.*t3.*t8.*t9.*t30.*t72.*1.724164458109665e-21;
et475 = t3.*t5.*t6.*t8.*t30.*t72.*(-7.690130037838559e-22);
et476 = t3.*t6.*t8.*t9.*t30.*t72.*(-4.179760421250838e-22);
et477 = 1.453096634654864e-3;
et478 = t90+t119+t150+t161-t168+t169-t172-t177+t1331-t1365+t1246.*(t965+t5.*(t531-t969)).*7.26350610236655e-5+t47.*t1249.*(t1289+t5.*(t649-t1220)).*1.015171749786156e-71;
et479 = t1249.*t1346.*(t26-t27).*5.517689141340903e-72;
et480 = t1249.*t1347.*(t26-t27).*1.015171749786156e-71;
et481 = t1342-t2.*t4.*t5.*5.463144604697158e-2;
et482 = t2.*t3.*t9.*9.189001945180305e-2;
et483 = t4.*t5.*t6.*1.324388487819695e-2;
et484 = t3.*t6.*t9.*(-2.227619671697157e-2);
et485 = t2.*t9.*t74.*1.324388487819695e-2;
et486 = t6.*t9.*t74.*5.463144604697158e-2;
et487 = t2.*t5.*t7.*t8.*9.189001945180305e-2;
et488 = t5.*t6.*t7.*t8.*(-2.227619671697157e-2);
et489 = t2.*t4.*t5.*t71.*2.227619671697157e-2;
et490 = t4.*t5.*t6.*t71.*9.189001945180305e-2;
et491 = t2.*t5.*t8.*t75.*1.324388487819695e-2;
et492 = t5.*t6.*t8.*t75.*5.463144604697158e-2-t2.*t7.*t9.*t30.*t72.*2.877233365226343e-18;
et493 = t6.*t7.*t9.*t30.*t72.*(-1.186867907736671e-17)+t2.*t3.*t5.*t8.*t30.*t72.*2.877233365226343e-18;
et494 = t3.*t5.*t6.*t8.*t30.*t72.*1.186867907736671e-17;
et495 = t1343-t2.*t3.*t5.*9.189001945180305e-2;
et496 = t3.*t5.*t6.*2.227619671697157e-2;
et497 = t2.*t4.*t9.*(-5.463144604697158e-2);
et498 = t4.*t6.*t9.*1.324388487819695e-2;
et499 = t2.*t5.*t74.*(-1.324388487819695e-2);
et500 = t5.*t6.*t74.*(-5.463144604697158e-2);
et501 = t2.*t7.*t8.*t9.*9.189001945180305e-2;
et502 = t6.*t7.*t8.*t9.*(-2.227619671697157e-2);
et503 = t2.*t4.*t9.*t71.*2.227619671697157e-2;
et504 = t4.*t6.*t9.*t71.*9.189001945180305e-2;
et505 = t2.*t8.*t9.*t75.*1.324388487819695e-2;
et506 = t6.*t8.*t9.*t75.*5.463144604697158e-2+t2.*t5.*t7.*t30.*t72.*2.877233365226343e-18;
et507 = t5.*t6.*t7.*t30.*t72.*1.186867907736671e-17+t2.*t3.*t8.*t9.*t30.*t72.*2.877233365226343e-18;
et508 = t3.*t6.*t8.*t9.*t30.*t72.*1.186867907736671e-17;
et509 = t1271-t2.*t4.*5.463144604697158e-2;
et510 = t4.*t6.*1.324388487819695e-2;
et511 = t2.*t7.*t8.*9.189001945180305e-2;
et512 = t6.*t7.*t8.*(-2.227619671697157e-2);
et513 = t2.*t4.*t71.*2.227619671697157e-2;
et514 = t4.*t6.*t71.*9.189001945180305e-2;
et515 = t2.*t8.*t75.*1.324388487819695e-2;
et516 = t6.*t8.*t75.*5.463144604697158e-2+t2.*t3.*t8.*t30.*t72.*2.877233365226343e-18;
et517 = t3.*t6.*t8.*t30.*t72.*1.186867907736671e-17;
et518 = t1245+t2.*t3.*9.189001945180305e-2;
et519 = t3.*t6.*(-2.227619671697157e-2);
et520 = t2.*t74.*1.324388487819695e-2+t6.*t74.*5.463144604697158e-2;
et521 = t2.*t7.*t30.*t72.*(-2.877233365226343e-18)-t6.*t7.*t30.*t72.*1.186867907736671e-17;
et522 = t380+t410+t581+t585+t588+t590+t593+t605-t617+t973-t1022-t1128+t1131-t1138-t1146-t1195-t1273+t1284+t1285-t1426+t1206.*(et478+et479+et480)+t1425.*(t965+t5.*(t531-t969))-t1204.*(t196+t200+t217+t219+t568+t570+t571+t572+t672+t674+t1272)-t1412.*(t196+t200+t217+t219+t568+t570+t571+t572+t672+t674+t1280)+t1419.*(et481+et482+et483+et484+et485+et486+et487+et488+et489+et490+et491+et492+et493+et494)-t1418.*(et495+et496+et497+et498+et499+et500+et501+et502+et503+et504+et505+et506+et507+et508);
et523 = t2.*t75.*4.3770347702589e-6;
et524 = t6.*t75.*1.805540754063641e-5-t1205.*(et509+et510+et511+et512+et513+et514+et515+et516+et517)+t1217.*(et518+et519+et520+et521);
et525 = t2.*t30.*t72.*(-2.751435409876806e-21);
et526 = t6.*t30.*t72.*(-1.134975851337029e-20);
et527 = t2.*t3.*t30.*t72.*2.483366197185125e-22;
et528 = t3.*t6.*t30.*t72.*1.024396449109444e-21;
K = dq1.*((dq2.*t1436)./2.0+(dq4.*t1435)./2.0+(dq5.*t1434)./2.0+(dq1.*(et406+et407+et408+et409+et410+et411+et412+et413+et414+et415+et416+et417+et418+et419+et420+et421+et422+et423+et424+et425+et426+et427+et428+et429+et430+et431+et432+et433+et434+et435+et436+et437+et438+et439+et440+et441+et442+et443+et444+et445+et446+et447+et448+et449+et450+et451+et452+et453+et454+et455+et456+et457+et458+et459+et460+et461+et462+et463+et464+et465+et466+et467+et468+et469+et470+et471+et472+et473+et474+et475+et476+et477))./2.0+(dq6.*(et402+et403+et404+et405))./2.0+(dq3.*(et522+et523+et524+et525+et526+et527+et528))./2.0)+et400.*et401+dq4.*(et22+et23)+dq2.*(et51+et52)+dq5.*(et81+et82)-dq3.*(et342+et343);
end
